simulink library "outp"  (R2021b)
(part 6 of 10)

      link override Signal_Override/_ovrdflg: Value=KOUTP_FDCBCMDVRSignalRCmd_flg_ovrdflg
      link override Signal_Override/_ovrdval: Value=KOUTP_FDCBCMDVRSignalRCmd_flg_ovrdval
  VBCM_FDCBCMEmExitSWSta_flg_Inproc : FVT_lib/outp/OverrideAndLimit  SystemSampleTime=-1  VariantActivationTime=update diagram  Latency=0  AutoFrameSizeCalculation=off
      link override Signal_Limit/_maxval: Value=KOUTP_FDCBCMEmExitSWSta_flg_maxval
      link override Signal_Limit/_minval: Value=KOUTP_FDCBCMEmExitSWSta_flg_minval
      link override Signal_Override/_ovrdflg: Value=KOUTP_FDCBCMEmExitSWSta_flg_ovrdflg
      link override Signal_Override/_ovrdval: Value=KOUTP_FDCBCMEmExitSWSta_flg_ovrdval
  VBCM_FDCBCMEmSVCmd_flg_Inproc : FVT_lib/outp/OverrideAndLimit  SystemSampleTime=-1  VariantActivationTime=update diagram  Latency=0  AutoFrameSizeCalculation=off
      link override Signal_Limit/_maxval: Value=KOUTP_FDCBCMEmSVCmd_flg_maxval
      link override Signal_Limit/_minval: Value=KOUTP_FDCBCMEmSVCmd_flg_minval
      link override Signal_Override/_ovrdflg: Value=KOUTP_FDCBCMEmSVCmd_flg_ovrdflg
      link override Signal_Override/_ovrdval: Value=KOUTP_FDCBCMEmSVCmd_flg_ovrdval
  VBCM_FDCBCMFDCloseSVCmd_flg_Inproc : FVT_lib/outp/OverrideAndLimit  SystemSampleTime=-1  VariantActivationTime=update diagram  Latency=0  AutoFrameSizeCalculation=off
      link override Signal_Limit/_maxval: Value=KOUTP_FDCBCMFDCloseSVCmd_flg_maxval
      link override Signal_Limit/_minval: Value=KOUTP_FDCBCMFDCloseSVCmd_flg_minval
      link override Signal_Override/_ovrdflg: Value=KOUTP_FDCBCMFDCloseSVCmd_flg_ovrdflg
      link override Signal_Override/_ovrdval: Value=KOUTP_FDCBCMFDCloseSVCmd_flg_ovrdval
  VBCM_FDCBCMFDOpenSVCmd_flg_Inproc : FVT_lib/outp/OverrideAndLimit  SystemSampleTime=-1  VariantActivationTime=update diagram  Latency=0  AutoFrameSizeCalculation=off
      link override Signal_Limit/_maxval: Value=KOUTP_FDCBCMFDOpenSVCmd_flg_maxval
      link override Signal_Limit/_minval: Value=KOUTP_FDCBCMFDOpenSVCmd_flg_minval
      link override Signal_Override/_ovrdflg: Value=KOUTP_FDCBCMFDOpenSVCmd_flg_ovrdflg
      link override Signal_Override/_ovrdval: Value=KOUTP_FDCBCMFDOpenSVCmd_flg_ovrdval
  VBCM_FDCBCMFDoorSta_flg_Inproc : FVT_lib/outp/OverrideAndLimit  SystemSampleTime=-1  VariantActivationTime=update diagram  Latency=0  AutoFrameSizeCalculation=off
      link override Signal_Limit/_maxval: Value=KOUTP_FDCBCMFDoorSta_flg_maxval
      link override Signal_Limit/_minval: Value=KOUTP_FDCBCMFDoorSta_flg_minval
      link override Signal_Override/_ovrdflg: Value=KOUTP_FDCBCMFDoorSta_flg_ovrdflg
      link override Signal_Override/_ovrdval: Value=KOUTP_FDCBCMFDoorSta_flg_ovrdval
  VBCM_FDCBCMFRoomLpCmd_pct_Inproc : FVT_lib/outp/OverrideAndLimit  SystemSampleTime=-1  VariantActivationTime=update diagram  Latency=0  AutoFrameSizeCalculation=off
      link override Signal_Limit/_maxval: Value=KOUTP_FDCBCMFRoomLpCmd_pct_maxval
      link override Signal_Limit/_minval: Value=KOUTP_FDCBCMFRoomLpCmd_pct_minval
      link override Signal_Override/_ovrdflg: Value=KOUTP_FDCBCMFRoomLpCmd_pct_ovrdflg
      link override Signal_Override/_ovrdval: Value=KOUTP_FDCBCMFRoomLpCmd_pct_ovrdval
  VBCM_FDCBCMFRoomLpSetSta_pct_Inproc : FVT_lib/outp/OverrideAndLimit  SystemSampleTime=-1  VariantActivationTime=update diagram  Latency=0  AutoFrameSizeCalculation=off
      link override Signal_Limit/_maxval: Value=KOUTP_FDCBCMFRoomLpSetSta_pct_maxval
      link override Signal_Limit/_minval: Value=KOUTP_FDCBCMFRoomLpSetSta_pct_minval
      link override Signal_Override/_ovrdflg: Value=KOUTP_FDCBCMFRoomLpSetSta_pct_ovrdflg
      link override Signal_Override/_ovrdval: Value=KOUTP_FDCBCMFRoomLpSetSta_pct_ovrdval
  VBCM_FDCBCMHBeamCmd_flg_Inproc : FVT_lib/outp/OverrideAndLimit  SystemSampleTime=-1  VariantActivationTime=update diagram  Latency=0  AutoFrameSizeCalculation=off
      link override Signal_Limit/_maxval: Value=KOUTP_FDCBCMHBeamCmd_flg_maxval
      link override Signal_Limit/_minval: Value=KOUTP_FDCBCMHBeamCmd_flg_minval
      link override Signal_Override/_ovrdflg: Value=KOUTP_FDCBCMHBeamCmd_flg_ovrdflg
      link override Signal_Override/_ovrdval: Value=KOUTP_FDCBCMHBeamCmd_flg_ovrdval
  VBCM_FDCBCMHelpINDCmd_flg_Inproc : FVT_lib/outp/OverrideAndLimit  SystemSampleTime=-1  VariantActivationTime=update diagram  Latency=0  AutoFrameSizeCalculation=off
      link override Signal_Limit/_maxval: Value=KOUTP_FDCBCMHelpINDCmd_flg_maxval
      link override Signal_Limit/_minval: Value=KOUTP_FDCBCMHelpINDCmd_flg_minval
      link override Signal_Override/_ovrdflg: Value=KOUTP_FDCBCMHelpINDCmd_flg_ovrdflg
      link override Signal_Override/_ovrdval: Value=KOUTP_FDCBCMHelpINDCmd_flg_ovrdval
  VBCM_FDCBCMInnerBuzzerCmd_flg_Inproc : FVT_lib/outp/OverrideAndLimit  SystemSampleTime=-1  VariantActivationTime=update diagram  Latency=0  AutoFrameSizeCalculation=off
      link override Signal_Limit/_maxval: Value=KOUTP_FDCBCMInnerBuzzerCmd_flg_maxval
      link override Signal_Limit/_minval: Value=KOUTP_FDCBCMInnerBuzzerCmd_flg_minval
      link override Signal_Override/_ovrdflg: Value=KOUTP_FDCBCMInnerBuzzerCmd_flg_ovrdflg
      link override Signal_Override/_ovrdval: Value=KOUTP_FDCBCMInnerBuzzerCmd_flg_ovrdval
  VBCM_FDCBCMInnerCallBellCmd_flg_Inproc : FVT_lib/outp/OverrideAndLimit  SystemSampleTime=-1  VariantActivationTime=update diagram  Latency=0  AutoFrameSizeCalculation=off
      link override Signal_Limit/_maxval: Value=KOUTP_FDCBCMInnerCallBellCmd_flg_maxval
      link override Signal_Limit/_minval: Value=KOUTP_FDCBCMInnerCallBellCmd_flg_minval
      link override Signal_Override/_ovrdflg: Value=KOUTP_FDCBCMInnerCallBellCmd_flg_ovrdflg
      link override Signal_Override/_ovrdval: Value=KOUTP_FDCBCMInnerCallBellCmd_flg_ovrdval
  VBCM_FDCBCMLBSDRCmd_flg_Inproc : FVT_lib/outp/OverrideAndLimit  SystemSampleTime=-1  VariantActivationTime=update diagram  Latency=0  AutoFrameSizeCalculation=off
      link override Signal_Limit/_maxval: Value=KOUTP_FDCBCMLBSDRCmd_flg_maxval
      link override Signal_Limit/_minval: Value=KOUTP_FDCBCMLBSDRCmd_flg_minval
      link override Signal_Override/_ovrdflg: Value=KOUTP_FDCBCMLBSDRCmd_flg_ovrdflg
      link override Signal_Override/_ovrdval: Value=KOUTP_FDCBCMLBSDRCmd_flg_ovrdval
  VBCM_FDCBCMLBSDYCmd_flg_Inproc : FVT_lib/outp/OverrideAndLimit  SystemSampleTime=-1  VariantActivationTime=update diagram  Latency=0  AutoFrameSizeCalculation=off
      link override Signal_Limit/_maxval: Value=KOUTP_FDCBCMLBSDYCmd_flg_maxval
      link override Signal_Limit/_minval: Value=KOUTP_FDCBCMLBSDYCmd_flg_minval
      link override Signal_Override/_ovrdflg: Value=KOUTP_FDCBCMLBSDYCmd_flg_ovrdflg
      link override Signal_Override/_ovrdval: Value=KOUTP_FDCBCMLBSDYCmd_flg_ovrdval
  VBCM_FDCBCMLBeamCmd_flg_Inproc : FVT_lib/outp/OverrideAndLimit  SystemSampleTime=-1  VariantActivationTime=update diagram  Latency=0  AutoFrameSizeCalculation=off
      link override Signal_Limit/_maxval: Value=KOUTP_FDCBCMLBeamCmd_flg_maxval
      link override Signal_Limit/_minval: Value=KOUTP_FDCBCMLBeamCmd_flg_minval
      link override Signal_Override/_ovrdflg: Value=KOUTP_FDCBCMLBeamCmd_flg_ovrdflg
      link override Signal_Override/_ovrdval: Value=KOUTP_FDCBCMLBeamCmd_flg_ovrdval
  VBCM_FDCBCMLDRLCmd_flg_Inproc : FVT_lib/outp/OverrideAndLimit  SystemSampleTime=-1  VariantActivationTime=update diagram  Latency=0  AutoFrameSizeCalculation=off
      link override Signal_Limit/_maxval: Value=KOUTP_FDCBCMLDRLCmd_flg_maxval
      link override Signal_Limit/_minval: Value=KOUTP_FDCBCMLDRLCmd_flg_minval
      link override Signal_Override/_ovrdflg: Value=KOUTP_FDCBCMLDRLCmd_flg_ovrdflg
      link override Signal_Override/_ovrdval: Value=KOUTP_FDCBCMLDRLCmd_flg_ovrdval
  VBCM_FDCBCMLTurnLpCmd_flg_Inproc : FVT_lib/outp/OverrideAndLimit  SystemSampleTime=-1  VariantActivationTime=update diagram  Latency=0  AutoFrameSizeCalculation=off
      link override Signal_Limit/_maxval: Value=KOUTP_FDCBCMLTurnLpCmd_flg_maxval
      link override Signal_Limit/_minval: Value=KOUTP_FDCBCMLTurnLpCmd_flg_minval
      link override Signal_Override/_ovrdflg: Value=KOUTP_FDCBCMLTurnLpCmd_flg_ovrdflg
      link override Signal_Override/_ovrdval: Value=KOUTP_FDCBCMLTurnLpCmd_flg_ovrdval
  VBCM_FDCBCMLTurnSWSta_flg_Inproc : FVT_lib/outp/OverrideAndLimit  SystemSampleTime=-1  VariantActivationTime=update diagram  Latency=0  AutoFrameSizeCalculation=off
      link override Signal_Limit/_maxval: Value=KOUTP_FDCBCMLTurnSWSta_flg_maxval
      link override Signal_Limit/_minval: Value=KOUTP_FDCBCMLTurnSWSta_flg_minval
      link override Signal_Override/_ovrdflg: Value=KOUTP_FDCBCMLTurnSWSta_flg_ovrdflg
      link override Signal_Override/_ovrdval: Value=KOUTP_FDCBCMLTurnSWSta_flg_ovrdval
  VBCM_FDCBCMMDCloseSVCmd_flg_Inproc : FVT_lib/outp/OverrideAndLimit  SystemSampleTime=-1  VariantActivationTime=update diagram  Latency=0  AutoFrameSizeCalculation=off
      link override Signal_Limit/_maxval: Value=KOUTP_FDCBCMMDCloseSVCmd_flg_maxval
      link override Signal_Limit/_minval: Value=KOUTP_FDCBCMMDCloseSVCmd_flg_minval
      link override Signal_Override/_ovrdflg: Value=KOUTP_FDCBCMMDCloseSVCmd_flg_ovrdflg
      link override Signal_Override/_ovrdval: Value=KOUTP_FDCBCMMDCloseSVCmd_flg_ovrdval
  VBCM_FDCBCMMDOpenSVCmd_flg_Inproc : FVT_lib/outp/OverrideAndLimit  SystemSampleTime=-1  VariantActivationTime=update diagram  Latency=0  AutoFrameSizeCalculation=off
      link override Signal_Limit/_maxval: Value=KOUTP_FDCBCMMDOpenSVCmd_flg_maxval
      link override Signal_Limit/_minval: Value=KOUTP_FDCBCMMDOpenSVCmd_flg_minval
      link override Signal_Override/_ovrdflg: Value=KOUTP_FDCBCMMDOpenSVCmd_flg_ovrdflg
      link override Signal_Override/_ovrdval: Value=KOUTP_FDCBCMMDOpenSVCmd_flg_ovrdval
  VBCM_FDCBCMMDoorSta_flg_Inproc : FVT_lib/outp/OverrideAndLimit  SystemSampleTime=-1  VariantActivationTime=update diagram  Latency=0  AutoFrameSizeCalculation=off
      link override Signal_Limit/_maxval: Value=KOUTP_FDCBCMMDoorSta_flg_maxval
      link override Signal_Limit/_minval: Value=KOUTP_FDCBCMMDoorSta_flg_minval
      link override Signal_Override/_ovrdflg: Value=KOUTP_FDCBCMMDoorSta_flg_ovrdflg
      link override Signal_Override/_ovrdval: Value=KOUTP_FDCBCMMDoorSta_flg_ovrdval
  VBCM_FDCBCMMRoomLpCmd_pct_Inproc : FVT_lib/outp/OverrideAndLimit  SystemSampleTime=-1  VariantActivationTime=update diagram  Latency=0  AutoFrameSizeCalculation=off
      link override Signal_Limit/_maxval: Value=KOUTP_FDCBCMMRoomLpCmd_pct_maxval
      link override Signal_Limit/_minval: Value=KOUTP_FDCBCMMRoomLpCmd_pct_minval
      link override Signal_Override/_ovrdflg: Value=KOUTP_FDCBCMMRoomLpCmd_pct_ovrdflg
      link override Signal_Override/_ovrdval: Value=KOUTP_FDCBCMMRoomLpCmd_pct_ovrdval
  VBCM_FDCBCMMRoomLpSetSta_pct_Inproc : FVT_lib/outp/OverrideAndLimit  SystemSampleTime=-1  VariantActivationTime=update diagram  Latency=0  AutoFrameSizeCalculation=off
      link override Signal_Limit/_maxval: Value=KOUTP_FDCBCMMRoomLpSetSta_pct_maxval
      link override Signal_Limit/_minval: Value=KOUTP_FDCBCMMRoomLpSetSta_pct_minval
      link override Signal_Override/_ovrdflg: Value=KOUTP_FDCBCMMRoomLpSetSta_pct_ovrdflg
      link override Signal_Override/_ovrdval: Value=KOUTP_FDCBCMMRoomLpSetSta_pct_ovrdval
  VBCM_FDCBCMOSDrOpenSWSta_enum_Inproc : FVT_lib/outp/OverrideAndLimit  SystemSampleTime=-1  VariantActivationTime=update diagram  Latency=0  AutoFrameSizeCalculation=off
      link override Signal_Limit/_maxval: Value=KOUTP_FDCBCMOSDrOpenSWSta_enum_maxval
      link override Signal_Limit/_minval: Value=KOUTP_FDCBCMOSDrOpenSWSta_enum_minval
      link override Signal_Override/_ovrdflg: Value=KOUTP_FDCBCMOSDrOpenSWSta_enum_ovrdflg
      link override Signal_Override/_ovrdval: Value=KOUTP_FDCBCMOSDrOpenSWSta_enum_ovrdval
  VBCM_FDCBCMPLampCmd_flg_Inproc : FVT_lib/outp/OverrideAndLimit  SystemSampleTime=-1  VariantActivationTime=update diagram  Latency=0  AutoFrameSizeCalculation=off
      link override Signal_Limit/_maxval: Value=KOUTP_FDCBCMPLampCmd_flg_maxval
      link override Signal_Limit/_minval: Value=KOUTP_FDCBCMPLampCmd_flg_minval
      link override Signal_Override/_ovrdflg: Value=KOUTP_FDCBCMPLampCmd_flg_ovrdflg
      link override Signal_Override/_ovrdval: Value=KOUTP_FDCBCMPLampCmd_flg_ovrdval
  VBCM_FDCBCMRBSDRCmd_flg_Inproc : FVT_lib/outp/OverrideAndLimit  SystemSampleTime=-1  VariantActivationTime=update diagram  Latency=0  AutoFrameSizeCalculation=off
      link override Signal_Limit/_maxval: Value=KOUTP_FDCBCMRBSDRCmd_flg_maxval
      link override Signal_Limit/_minval: Value=KOUTP_FDCBCMRBSDRCmd_flg_minval
      link override Signal_Override/_ovrdflg: Value=KOUTP_FDCBCMRBSDRCmd_flg_ovrdflg
      link override Signal_Override/_ovrdval: Value=KOUTP_FDCBCMRBSDRCmd_flg_ovrdval
  VBCM_FDCBCMRBSDYCmd_flg_Inproc : FVT_lib/outp/OverrideAndLimit  SystemSampleTime=-1  VariantActivationTime=update diagram  Latency=0  AutoFrameSizeCalculation=off
      link override Signal_Limit/_maxval: Value=KOUTP_FDCBCMRBSDYCmd_flg_maxval
      link override Signal_Limit/_minval: Value=KOUTP_FDCBCMRBSDYCmd_flg_minval
      link override Signal_Override/_ovrdflg: Value=KOUTP_FDCBCMRBSDYCmd_flg_ovrdflg
      link override Signal_Override/_ovrdval: Value=KOUTP_FDCBCMRBSDYCmd_flg_ovrdval
  VBCM_FDCBCMRDRLCmd_flg_Inproc : FVT_lib/outp/OverrideAndLimit  SystemSampleTime=-1  VariantActivationTime=update diagram  Latency=0  AutoFrameSizeCalculation=off
      link override Signal_Limit/_maxval: Value=KOUTP_FDCBCMRDRLCmd_flg_maxval
      link override Signal_Limit/_minval: Value=KOUTP_FDCBCMRDRLCmd_flg_minval
      link override Signal_Override/_ovrdflg: Value=KOUTP_FDCBCMRDRLCmd_flg_ovrdflg
      link override Signal_Override/_ovrdval: Value=KOUTP_FDCBCMRDRLCmd_flg_ovrdval
  VBCM_FDCBCMRDoorSta_flg_Inproc : FVT_lib/outp/OverrideAndLimit  SystemSampleTime=-1  VariantActivationTime=update diagram  Latency=0  AutoFrameSizeCalculation=off
      link override Signal_Limit/_maxval: Value=KOUTP_FDCBCMRDoorSta_flg_maxval
      link override Signal_Limit/_minval: Value=KOUTP_FDCBCMRDoorSta_flg_minval
      link override Signal_Override/_ovrdflg: Value=KOUTP_FDCBCMRDoorSta_flg_ovrdflg
      link override Signal_Override/_ovrdval: Value=KOUTP_FDCBCMRDoorSta_flg_ovrdval
  VBCM_FDCBCMRFLampCmd_flg_Inproc : FVT_lib/outp/OverrideAndLimit  SystemSampleTime=-1  VariantActivationTime=update diagram  Latency=0  AutoFrameSizeCalculation=off
      link override Signal_Limit/_maxval: Value=KOUTP_FDCBCMRFLampCmd_flg_maxval
      link override Signal_Limit/_minval: Value=KOUTP_FDCBCMRFLampCmd_flg_minval
      link override Signal_Override/_ovrdflg: Value=KOUTP_FDCBCMRFLampCmd_flg_ovrdflg
      link override Signal_Override/_ovrdval: Value=KOUTP_FDCBCMRFLampCmd_flg_ovrdval
  VBCM_FDCBCMRGearSta_flg_Inproc : FVT_lib/outp/OverrideAndLimit  SystemSampleTime=-1  VariantActivationTime=update diagram  Latency=0  AutoFrameSizeCalculation=off
      link override Signal_Limit/_maxval: Value=KOUTP_FDCBCMRGearSta_flg_maxval
      link override Signal_Limit/_minval: Value=KOUTP_FDCBCMRGearSta_flg_minval
      link override Signal_Override/_ovrdflg: Value=KOUTP_FDCBCMRGearSta_flg_ovrdflg
      link override Signal_Override/_ovrdval: Value=KOUTP_FDCBCMRGearSta_flg_ovrdval
  VBCM_FDCBCMRRoomLpCmd_pct_Inproc : FVT_lib/outp/OverrideAndLimit  SystemSampleTime=-1  VariantActivationTime=update diagram  Latency=0  AutoFrameSizeCalculation=off
      link override Signal_Limit/_maxval: Value=KOUTP_FDCBCMRRoomLpCmd_pct_maxval
      link override Signal_Limit/_minval: Value=KOUTP_FDCBCMRRoomLpCmd_pct_minval
      link override Signal_Override/_ovrdflg: Value=KOUTP_FDCBCMRRoomLpCmd_pct_ovrdflg
      link override Signal_Override/_ovrdval: Value=KOUTP_FDCBCMRRoomLpCmd_pct_ovrdval
  VBCM_FDCBCMRRoomLpSetSta_pct_Inproc : FVT_lib/outp/OverrideAndLimit  SystemSampleTime=-1  VariantActivationTime=update diagram  Latency=0  AutoFrameSizeCalculation=off
      link override Signal_Limit/_maxval: Value=KOUTP_FDCBCMRRoomLpSetSta_pct_maxval
      link override Signal_Limit/_minval: Value=KOUTP_FDCBCMRRoomLpSetSta_pct_minval
      link override Signal_Override/_ovrdflg: Value=KOUTP_FDCBCMRRoomLpSetSta_pct_ovrdflg
      link override Signal_Override/_ovrdval: Value=KOUTP_FDCBCMRRoomLpSetSta_pct_ovrdval
  VBCM_FDCBCMRTurnLpCmd_flg_Inproc : FVT_lib/outp/OverrideAndLimit  SystemSampleTime=-1  VariantActivationTime=update diagram  Latency=0  AutoFrameSizeCalculation=off
      link override Signal_Limit/_maxval: Value=KOUTP_FDCBCMRTurnLpCmd_flg_maxval
      link override Signal_Limit/_minval: Value=KOUTP_FDCBCMRTurnLpCmd_flg_minval
      link override Signal_Override/_ovrdflg: Value=KOUTP_FDCBCMRTurnLpCmd_flg_ovrdflg
      link override Signal_Override/_ovrdval: Value=KOUTP_FDCBCMRTurnLpCmd_flg_ovrdval
  VBCM_FDCBCMRTurnSWSta_flg_Inproc : FVT_lib/outp/OverrideAndLimit  SystemSampleTime=-1  VariantActivationTime=update diagram  Latency=0  AutoFrameSizeCalculation=off
      link override Signal_Limit/_maxval: Value=KOUTP_FDCBCMRTurnSWSta_flg_maxval
      link override Signal_Limit/_minval: Value=KOUTP_FDCBCMRTurnSWSta_flg_minval
      link override Signal_Override/_ovrdflg: Value=KOUTP_FDCBCMRTurnSWSta_flg_ovrdflg
      link override Signal_Override/_ovrdval: Value=KOUTP_FDCBCMRTurnSWSta_flg_ovrdval
  VBCM_FDCBCMRoomLpAmbCmd_flg_Inproc : FVT_lib/outp/OverrideAndLimit  SystemSampleTime=-1  VariantActivationTime=update diagram  Latency=0  AutoFrameSizeCalculation=off
      link override Signal_Limit/_maxval: Value=KOUTP_FDCBCMRoomLpAmbCmd_flg_maxval
      link override Signal_Limit/_minval: Value=KOUTP_FDCBCMRoomLpAmbCmd_flg_minval
      link override Signal_Override/_ovrdflg: Value=KOUTP_FDCBCMRoomLpAmbCmd_flg_ovrdflg
      link override Signal_Override/_ovrdval: Value=KOUTP_FDCBCMRoomLpAmbCmd_flg_ovrdval
  VBCM_FDCBCMRoomLpAmbSetSta_flg_Inproc : FVT_lib/outp/OverrideAndLimit  SystemSampleTime=-1  VariantActivationTime=update diagram  Latency=0  AutoFrameSizeCalculation=off
      link override Signal_Limit/_maxval: Value=KOUTP_FDCBCMRoomLpAmbSetSta_flg_maxval
      link override Signal_Limit/_minval: Value=KOUTP_FDCBCMRoomLpAmbSetSta_flg_minval
      link override Signal_Override/_ovrdflg: Value=KOUTP_FDCBCMRoomLpAmbSetSta_flg_ovrdflg
      link override Signal_Override/_ovrdval: Value=KOUTP_FDCBCMRoomLpAmbSetSta_flg_ovrdval
  VBCM_FDCBCMRoomLpSetSta_flg_Inproc : FVT_lib/outp/OverrideAndLimit  SystemSampleTime=-1  VariantActivationTime=update diagram  Latency=0  AutoFrameSizeCalculation=off
      link override Signal_Limit/_maxval: Value=KOUTP_FDCBCMRoomLpSetSta_flg_maxval
      link override Signal_Limit/_minval: Value=KOUTP_FDCBCMRoomLpSetSta_flg_minval
      link override Signal_Override/_ovrdflg: Value=KOUTP_FDCBCMRoomLpSetSta_flg_ovrdflg
      link override Signal_Override/_ovrdval: Value=KOUTP_FDCBCMRoomLpSetSta_flg_ovrdval
  VBCM_FDCBCMSLTLpCmd_flg_Inproc : FVT_lib/outp/OverrideAndLimit  SystemSampleTime=-1  VariantActivationTime=update diagram  Latency=0  AutoFrameSizeCalculation=off
      link override Signal_Limit/_maxval: Value=KOUTP_FDCBCMSLTLpCmd_flg_maxval
      link override Signal_Limit/_minval: Value=KOUTP_FDCBCMSLTLpCmd_flg_minval
      link override Signal_Override/_ovrdflg: Value=KOUTP_FDCBCMSLTLpCmd_flg_ovrdflg
      link override Signal_Override/_ovrdval: Value=KOUTP_FDCBCMSLTLpCmd_flg_ovrdval
  VBCM_FDCBCMSMKLCmd_flg_Inproc : FVT_lib/outp/OverrideAndLimit  SystemSampleTime=-1  VariantActivationTime=update diagram  Latency=0  AutoFrameSizeCalculation=off
      link override Signal_Limit/_maxval: Value=KOUTP_FDCBCMSMKLCmd_flg_maxval
      link override Signal_Limit/_minval: Value=KOUTP_FDCBCMSMKLCmd_flg_minval
      link override Signal_Override/_ovrdflg: Value=KOUTP_FDCBCMSMKLCmd_flg_ovrdflg
      link override Signal_Override/_ovrdval: Value=KOUTP_FDCBCMSMKLCmd_flg_ovrdval
  VBCM_FDCBCMSMKRCmd_flg_Inproc : FVT_lib/outp/OverrideAndLimit  SystemSampleTime=-1  VariantActivationTime=update diagram  Latency=0  AutoFrameSizeCalculation=off
      link override Signal_Limit/_maxval: Value=KOUTP_FDCBCMSMKRCmd_flg_maxval
      link override Signal_Limit/_minval: Value=KOUTP_FDCBCMSMKRCmd_flg_minval
      link override Signal_Override/_ovrdflg: Value=KOUTP_FDCBCMSMKRCmd_flg_ovrdflg
      link override Signal_Override/_ovrdval: Value=KOUTP_FDCBCMSMKRCmd_flg_ovrdval
  VBCM_FDCBCMSRTLpCmd_flg_Inproc : FVT_lib/outp/OverrideAndLimit  SystemSampleTime=-1  VariantActivationTime=update diagram  Latency=0  AutoFrameSizeCalculation=off
      link override Signal_Limit/_maxval: Value=KOUTP_FDCBCMSRTLpCmd_flg_maxval
      link override Signal_Limit/_minval: Value=KOUTP_FDCBCMSRTLpCmd_flg_minval
      link override Signal_Override/_ovrdflg: Value=KOUTP_FDCBCMSRTLpCmd_flg_ovrdflg
      link override Signal_Override/_ovrdval: Value=KOUTP_FDCBCMSRTLpCmd_flg_ovrdval
  VBCM_FDCBCMSTOPBALLCmd_flg_Inproc : FVT_lib/outp/OverrideAndLimit  SystemSampleTime=-1  VariantActivationTime=update diagram  Latency=0  AutoFrameSizeCalculation=off
      link override Signal_Limit/_maxval: Value=KOUTP_FDCBCMSTOPBALLCmd_flg_maxval
      link override Signal_Limit/_minval: Value=KOUTP_FDCBCMSTOPBALLCmd_flg_minval
      link override Signal_Override/_ovrdflg: Value=KOUTP_FDCBCMSTOPBALLCmd_flg_ovrdflg
      link override Signal_Override/_ovrdval: Value=KOUTP_FDCBCMSTOPBALLCmd_flg_ovrdval
  VBCM_FDCBCMStopINDCmd_flg_Inproc : FVT_lib/outp/OverrideAndLimit  SystemSampleTime=-1  VariantActivationTime=update diagram  Latency=0  AutoFrameSizeCalculation=off
      link override Signal_Limit/_maxval: Value=KOUTP_FDCBCMStopINDCmd_flg_maxval
      link override Signal_Limit/_minval: Value=KOUTP_FDCBCMStopINDCmd_flg_minval
      link override Signal_Override/_ovrdflg: Value=KOUTP_FDCBCMStopINDCmd_flg_ovrdflg
      link override Signal_Override/_ovrdval: Value=KOUTP_FDCBCMStopINDCmd_flg_ovrdval
  VBCM_FDCBCMTurnBuzzerENSta_flg_Inproc : FVT_lib/outp/OverrideAndLimit  SystemSampleTime=-1  VariantActivationTime=update diagram  Latency=0  AutoFrameSizeCalculation=off
      link override Signal_Limit/_maxval: Value=KOUTP_FDCBCMTurnBuzzerENSta_flg_maxval
      link override Signal_Limit/_minval: Value=KOUTP_FDCBCMTurnBuzzerENSta_flg_minval
      link override Signal_Override/_ovrdflg: Value=KOUTP_FDCBCMTurnBuzzerENSta_flg_ovrdflg
      link override Signal_Override/_ovrdval: Value=KOUTP_FDCBCMTurnBuzzerENSta_flg_ovrdval
  VBCM_FDCBCMWasherCmd_flg_Inproc : FVT_lib/outp/OverrideAndLimit  SystemSampleTime=-1  VariantActivationTime=update diagram  Latency=0  AutoFrameSizeCalculation=off
      link override Signal_Limit/_maxval: Value=KOUTP_FDCBCMWasherCmd_flg_maxval
      link override Signal_Limit/_minval: Value=KOUTP_FDCBCMWasherCmd_flg_minval
      link override Signal_Override/_ovrdflg: Value=KOUTP_FDCBCMWasherCmd_flg_ovrdflg
      link override Signal_Override/_ovrdval: Value=KOUTP_FDCBCMWasherCmd_flg_ovrdval
  VBCM_FDCBCMWiperHCmd_flg_Inproc : FVT_lib/outp/OverrideAndLimit  SystemSampleTime=-1  VariantActivationTime=update diagram  Latency=0  AutoFrameSizeCalculation=off
      link override Signal_Limit/_maxval: Value=KOUTP_FDCBCMWiperHCmd_flg_maxval
      link override Signal_Limit/_minval: Value=KOUTP_FDCBCMWiperHCmd_flg_minval
      link override Signal_Override/_ovrdflg: Value=KOUTP_FDCBCMWiperHCmd_flg_ovrdflg
      link override Signal_Override/_ovrdval: Value=KOUTP_FDCBCMWiperHCmd_flg_ovrdval
  VBCM_FDCBCMWiperLCmd_flg_Inproc : FVT_lib/outp/OverrideAndLimit  SystemSampleTime=-1  VariantActivationTime=update diagram  Latency=0  AutoFrameSizeCalculation=off
      link override Signal_Limit/_maxval: Value=KOUTP_FDCBCMWiperLCmd_flg_maxval
      link override Signal_Limit/_minval: Value=KOUTP_FDCBCMWiperLCmd_flg_minval
      link override Signal_Override/_ovrdflg: Value=KOUTP_FDCBCMWiperLCmd_flg_ovrdflg
      link override Signal_Override/_ovrdval: Value=KOUTP_FDCBCMWiperLCmd_flg_ovrdval
  VBCM_InnerBuzzerModeSta_enum_Inproc : FVT_lib/outp/OverrideAndLimit  SystemSampleTime=-1  VariantActivationTime=update diagram  Latency=0  AutoFrameSizeCalculation=off
      link override Signal_Limit/_maxval: Value=KOUTP_InnerBuzzerModeSta_enum_maxval
      link override Signal_Limit/_minval: Value=KOUTP_InnerBuzzerModeSta_enum_minval
      link override Signal_Override/_ovrdflg: Value=KOUTP_InnerBuzzerModeSta_enum_ovrdflg
      link override Signal_Override/_ovrdval: Value=KOUTP_InnerBuzzerModeSta_enum_ovrdval
  VBCM_KeepWakeUp_flg_Inproc : FVT_lib/outp/OverrideAndLimit  SystemSampleTime=-1  VariantActivationTime=update diagram  Latency=0  AutoFrameSizeCalculation=off
      link override Signal_Limit/_maxval: Value=KOUTP_KeepWakeUp_flg_maxval
      link override Signal_Limit/_minval: Value=KOUTP_KeepWakeUp_flg_minval
      link override Signal_Override/_ovrdflg: Value=KOUTP_KeepWakeUp_flg_ovrdflg
      link override Signal_Override/_ovrdval: Value=KOUTP_KeepWakeUp_flg_ovrdval
  VBCM_TurnLpPatternSta_enum_Inproc : FVT_lib/outp/OverrideAndLimit  SystemSampleTime=-1  VariantActivationTime=update diagram  Latency=0  AutoFrameSizeCalculation=off
      link override Signal_Limit/_maxval: Value=KOUTP_TurnLpPatternSta_enum_maxval
      link override Signal_Limit/_minval: Value=KOUTP_TurnLpPatternSta_enum_minval
      link override Signal_Override/_ovrdflg: Value=KOUTP_TurnLpPatternSta_enum_ovrdflg
      link override Signal_Override/_ovrdval: Value=KOUTP_TurnLpPatternSta_enum_ovrdval
  VBCM_WakeUp_flg_Inproc : FVT_lib/outp/OverrideAndLimit  SystemSampleTime=-1  VariantActivationTime=update diagram  Latency=0  AutoFrameSizeCalculation=off
      link override Signal_Limit/_maxval: Value=KOUTP_WakeUp_flg_maxval
      link override Signal_Limit/_minval: Value=KOUTP_WakeUp_flg_minval
      link override Signal_Override/_ovrdflg: Value=KOUTP_WakeUp_flg_ovrdflg
      link override Signal_Override/_ovrdval: Value=KOUTP_WakeUp_flg_ovrdval
  VDDM_5vAPS1PwrErrDTC_raw32_Inproc : FVT_lib/outp/OverrideAndLimit  SystemSampleTime=-1  VariantActivationTime=update diagram  Latency=0  AutoFrameSizeCalculation=off
      link override Signal_Limit/_maxval: Value=KOUTP_5vAPS1PwrErrDTC_raw32_maxval
      link override Signal_Limit/_minval: Value=KOUTP_5vAPS1PwrErrDTC_raw32_minval
      link override Signal_Override/_ovrdflg: Value=KOUTP_5vAPS1PwrErrDTC_raw32_ovrdflg
      link override Signal_Override/_ovrdval: Value=KOUTP_5vAPS1PwrErrDTC_raw32_ovrdval
  VDDM_5vAPS2PwrErrDTC_raw32_Inproc : FVT_lib/outp/OverrideAndLimit  SystemSampleTime=-1  VariantActivationTime=update diagram  Latency=0  AutoFrameSizeCalculation=off
      link override Signal_Limit/_maxval: Value=KOUTP_5vAPS2PwrErrDTC_raw32_maxval
      link override Signal_Limit/_minval: Value=KOUTP_5vAPS2PwrErrDTC_raw32_minval
      link override Signal_Override/_ovrdflg: Value=KOUTP_5vAPS2PwrErrDTC_raw32_ovrdflg
      link override Signal_Override/_ovrdval: Value=KOUTP_5vAPS2PwrErrDTC_raw32_ovrdval
  VDDM_ACCAccelCmdErrDetDTC_raw32_Inproc : FVT_lib/outp/OverrideAndLimit  SystemSampleTime=-1  VariantActivationTime=update diagram  Latency=0  AutoFrameSizeCalculation=off
      link override Signal_Limit/_maxval: Value=KOUTP_ACCAccelCmdErrDetDTC_raw32_maxval
      link override Signal_Limit/_minval: Value=KOUTP_ACCAccelCmdErrDetDTC_raw32_minval
      link override Signal_Override/_ovrdflg: Value=KOUTP_ACCAccelCmdErrDetDTC_raw32_ovrdflg
      link override Signal_Override/_ovrdval: Value=KOUTP_ACCAccelCmdErrDetDTC_raw32_ovrdval
  VDDM_ACCMalfuncDetDTC_raw32_Inproc : FVT_lib/outp/OverrideAndLimit  SystemSampleTime=-1  VariantActivationTime=update diagram  Latency=0  AutoFrameSizeCalculation=off
      link override Signal_Limit/_maxval: Value=KOUTP_ACCMalfuncDetDTC_raw32_maxval
      link override Signal_Limit/_minval: Value=KOUTP_ACCMalfuncDetDTC_raw32_minval
      link override Signal_Override/_ovrdflg: Value=KOUTP_ACCMalfuncDetDTC_raw32_ovrdflg
      link override Signal_Override/_ovrdval: Value=KOUTP_ACCMalfuncDetDTC_raw32_ovrdval
  VDDM_APS1SigOoRDTC_raw32_Inproc : FVT_lib/outp/OverrideAndLimit  SystemSampleTime=-1  VariantActivationTime=update diagram  Latency=0  AutoFrameSizeCalculation=off
      link override Signal_Limit/_maxval: Value=KOUTP_APS1SigOoRDTC_raw32_maxval
      link override Signal_Limit/_minval: Value=KOUTP_APS1SigOoRDTC_raw32_minval
      link override Signal_Override/_ovrdflg: Value=KOUTP_APS1SigOoRDTC_raw32_ovrdflg
      link override Signal_Override/_ovrdval: Value=KOUTP_APS1SigOoRDTC_raw32_ovrdval
  VDDM_APS2SigOoRDTC_raw32_Inproc : FVT_lib/outp/OverrideAndLimit  SystemSampleTime=-1  VariantActivationTime=update diagram  Latency=0  AutoFrameSizeCalculation=off
      link override Signal_Limit/_maxval: Value=KOUTP_APS2SigOoRDTC_raw32_maxval
      link override Signal_Limit/_minval: Value=KOUTP_APS2SigOoRDTC_raw32_minval
      link override Signal_Override/_ovrdflg: Value=KOUTP_APS2SigOoRDTC_raw32_ovrdflg
      link override Signal_Override/_ovrdval: Value=KOUTP_APS2SigOoRDTC_raw32_ovrdval
  VDDM_APSCorrErrDTC_raw32_Inproc : FVT_lib/outp/OverrideAndLimit  SystemSampleTime=-1  VariantActivationTime=update diagram  Latency=0  AutoFrameSizeCalculation=off
      link override Signal_Limit/_maxval: Value=KOUTP_APSCorrErrDTC_raw32_maxval
      link override Signal_Limit/_minval: Value=KOUTP_APSCorrErrDTC_raw32_minval
      link override Signal_Override/_ovrdflg: Value=KOUTP_APSCorrErrDTC_raw32_ovrdflg
      link override Signal_Override/_ovrdval: Value=KOUTP_APSCorrErrDTC_raw32_ovrdval
  VDDM_BMSRdyDTC_raw32_Inproc : FVT_lib/outp/OverrideAndLimit  SystemSampleTime=-1  VariantActivationTime=update diagram  Latency=0  AutoFrameSizeCalculation=off
      link override Signal_Limit/_maxval: Value=KOUTP_BMSRdyDTC_raw32_maxval
      link override Signal_Limit/_minval: Value=KOUTP_BMSRdyDTC_raw32_minval
      link override Signal_Override/_ovrdflg: Value=KOUTP_BMSRdyDTC_raw32_ovrdflg
      link override Signal_Override/_ovrdval: Value=KOUTP_BMSRdyDTC_raw32_ovrdval
  VDDM_BMSSigErrDetDTC_raw32_Inproc : FVT_lib/outp/OverrideAndLimit  SystemSampleTime=-1  VariantActivationTime=update diagram  Latency=0  AutoFrameSizeCalculation=off
      link override Signal_Limit/_maxval: Value=KOUTP_BMSSigErrDetDTC_raw32_maxval
      link override Signal_Limit/_minval: Value=KOUTP_BMSSigErrDetDTC_raw32_minval
      link override Signal_Override/_ovrdflg: Value=KOUTP_BMSSigErrDetDTC_raw32_ovrdflg
      link override Signal_Override/_ovrdval: Value=KOUTP_BMSSigErrDetDTC_raw32_ovrdval
  VDDM_BrkSWErrDTC_raw32_Inproc : FVT_lib/outp/OverrideAndLimit  SystemSampleTime=-1  VariantActivationTime=update diagram  Latency=0  AutoFrameSizeCalculation=off
      link override Signal_Limit/_maxval: Value=KOUTP_BrkSWErrDTC_raw32_maxval
      link override Signal_Limit/_minval: Value=KOUTP_BrkSWErrDTC_raw32_minval
      link override Signal_Override/_ovrdflg: Value=KOUTP_BrkSWErrDTC_raw32_ovrdflg
      link override Signal_Override/_ovrdval: Value=KOUTP_BrkSWErrDTC_raw32_ovrdval
  VDDM_BrkSWNoBacDTC_raw32_Inproc : FVT_lib/outp/OverrideAndLimit  SystemSampleTime=-1  VariantActivationTime=update diagram  Latency=0  AutoFrameSizeCalculation=off
      link override Signal_Limit/_maxval: Value=KOUTP_BrkSWNoBacDTC_raw32_maxval
      link override Signal_Limit/_minval: Value=KOUTP_BrkSWNoBacDTC_raw32_minval
      link override Signal_Override/_ovrdflg: Value=KOUTP_BrkSWNoBacDTC_raw32_ovrdflg
      link override Signal_Override/_ovrdval: Value=KOUTP_BrkSWNoBacDTC_raw32_ovrdval
  VDDM_C1ABM1CSDTC_raw32_Inproc : FVT_lib/outp/OverrideAndLimit  SystemSampleTime=-1  VariantActivationTime=update diagram  Latency=0  AutoFrameSizeCalculation=off
      link override Signal_Limit/_maxval: Value=KOUTP_C1ABM1CSDTC_raw32_maxval
      link override Signal_Limit/_minval: Value=KOUTP_C1ABM1CSDTC_raw32_minval
      link override Signal_Override/_ovrdflg: Value=KOUTP_C1ABM1CSDTC_raw32_ovrdflg
      link override Signal_Override/_ovrdval: Value=KOUTP_C1ABM1CSDTC_raw32_ovrdval
  VDDM_C1ABM1LCDTC_raw32_Inproc : FVT_lib/outp/OverrideAndLimit  SystemSampleTime=-1  VariantActivationTime=update diagram  Latency=0  AutoFrameSizeCalculation=off
      link override Signal_Limit/_maxval: Value=KOUTP_C1ABM1LCDTC_raw32_maxval
      link override Signal_Limit/_minval: Value=KOUTP_C1ABM1LCDTC_raw32_minval
      link override Signal_Override/_ovrdflg: Value=KOUTP_C1ABM1LCDTC_raw32_ovrdflg
      link override Signal_Override/_ovrdval: Value=KOUTP_C1ABM1LCDTC_raw32_ovrdval
  VDDM_C1ABM1RCDTC_raw32_Inproc : FVT_lib/outp/OverrideAndLimit  SystemSampleTime=-1  VariantActivationTime=update diagram  Latency=0  AutoFrameSizeCalculation=off
      link override Signal_Limit/_maxval: Value=KOUTP_C1ABM1RCDTC_raw32_maxval
      link override Signal_Limit/_minval: Value=KOUTP_C1ABM1RCDTC_raw32_minval
      link override Signal_Override/_ovrdflg: Value=KOUTP_C1ABM1RCDTC_raw32_ovrdflg
      link override Signal_Override/_ovrdval: Value=KOUTP_C1ABM1RCDTC_raw32_ovrdval
  VDDM_C1EPAS2LCDTC_raw32_Inproc : FVT_lib/outp/OverrideAndLimit  SystemSampleTime=-1  VariantActivationTime=update diagram  Latency=0  AutoFrameSizeCalculation=off
      link override Signal_Limit/_maxval: Value=KOUTP_C1EPAS2LCDTC_raw32_maxval
      link override Signal_Limit/_minval: Value=KOUTP_C1EPAS2LCDTC_raw32_minval
      link override Signal_Override/_ovrdflg: Value=KOUTP_C1EPAS2LCDTC_raw32_ovrdflg
      link override Signal_Override/_ovrdval: Value=KOUTP_C1EPAS2LCDTC_raw32_ovrdval
  VDDM_C3BMS1CSDTC_raw32_Inproc : FVT_lib/outp/OverrideAndLimit  SystemSampleTime=-1  VariantActivationTime=update diagram  Latency=0  AutoFrameSizeCalculation=off
      link override Signal_Limit/_maxval: Value=KOUTP_C3BMS1CSDTC_raw32_maxval
      link override Signal_Limit/_minval: Value=KOUTP_C3BMS1CSDTC_raw32_minval
      link override Signal_Override/_ovrdflg: Value=KOUTP_C3BMS1CSDTC_raw32_ovrdflg
      link override Signal_Override/_ovrdval: Value=KOUTP_C3BMS1CSDTC_raw32_ovrdval
  VDDM_C3BMS1LCDTC_raw32_Inproc : FVT_lib/outp/OverrideAndLimit  SystemSampleTime=-1  VariantActivationTime=update diagram  Latency=0  AutoFrameSizeCalculation=off
      link override Signal_Limit/_maxval: Value=KOUTP_C3BMS1LCDTC_raw32_maxval
      link override Signal_Limit/_minval: Value=KOUTP_C3BMS1LCDTC_raw32_minval
      link override Signal_Override/_ovrdflg: Value=KOUTP_C3BMS1LCDTC_raw32_ovrdflg
      link override Signal_Override/_ovrdval: Value=KOUTP_C3BMS1LCDTC_raw32_ovrdval
  VDDM_C3BMS1RCDTC_raw32_Inproc : FVT_lib/outp/OverrideAndLimit  SystemSampleTime=-1  VariantActivationTime=update diagram  Latency=0  AutoFrameSizeCalculation=off
      link override Signal_Limit/_maxval: Value=KOUTP_C3BMS1RCDTC_raw32_maxval
      link override Signal_Limit/_minval: Value=KOUTP_C3BMS1RCDTC_raw32_minval
      link override Signal_Override/_ovrdflg: Value=KOUTP_C3BMS1RCDTC_raw32_ovrdflg
      link override Signal_Override/_ovrdval: Value=KOUTP_C3BMS1RCDTC_raw32_ovrdval
  VDDM_C3BMS6CSDTC_raw32_Inproc : FVT_lib/outp/OverrideAndLimit  SystemSampleTime=-1  VariantActivationTime=update diagram  Latency=0  AutoFrameSizeCalculation=off
      link override Signal_Limit/_maxval: Value=KOUTP_C3BMS6CSDTC_raw32_maxval
      link override Signal_Limit/_minval: Value=KOUTP_C3BMS6CSDTC_raw32_minval
      link override Signal_Override/_ovrdflg: Value=KOUTP_C3BMS6CSDTC_raw32_ovrdflg
      link override Signal_Override/_ovrdval: Value=KOUTP_C3BMS6CSDTC_raw32_ovrdval
  VDDM_C3BMS6LCDTC_raw32_Inproc : FVT_lib/outp/OverrideAndLimit  SystemSampleTime=-1  VariantActivationTime=update diagram  Latency=0  AutoFrameSizeCalculation=off
      link override Signal_Limit/_maxval: Value=KOUTP_C3BMS6LCDTC_raw32_maxval
      link override Signal_Limit/_minval: Value=KOUTP_C3BMS6LCDTC_raw32_minval
      link override Signal_Override/_ovrdflg: Value=KOUTP_C3BMS6LCDTC_raw32_ovrdflg
      link override Signal_Override/_ovrdval: Value=KOUTP_C3BMS6LCDTC_raw32_ovrdval
  VDDM_C3BMS6RCDTC_raw32_Inproc : FVT_lib/outp/OverrideAndLimit  SystemSampleTime=-1  VariantActivationTime=update diagram  Latency=0  AutoFrameSizeCalculation=off
      link override Signal_Limit/_maxval: Value=KOUTP_C3BMS6RCDTC_raw32_maxval
      link override Signal_Limit/_minval: Value=KOUTP_C3BMS6RCDTC_raw32_minval
      link override Signal_Override/_ovrdflg: Value=KOUTP_C3BMS6RCDTC_raw32_ovrdflg
      link override Signal_Override/_ovrdval: Value=KOUTP_C3BMS6RCDTC_raw32_ovrdval
  VDDM_C3CCU1CSDTC_raw32_Inproc : FVT_lib/outp/OverrideAndLimit  SystemSampleTime=-1  VariantActivationTime=update diagram  Latency=0  AutoFrameSizeCalculation=off
      link override Signal_Limit/_maxval: Value=KOUTP_C3CCU1CSDTC_raw32_maxval
      link override Signal_Limit/_minval: Value=KOUTP_C3CCU1CSDTC_raw32_minval
      link override Signal_Override/_ovrdflg: Value=KOUTP_C3CCU1CSDTC_raw32_ovrdflg
      link override Signal_Override/_ovrdval: Value=KOUTP_C3CCU1CSDTC_raw32_ovrdval
  VDDM_C3CCU1LCDTC_raw32_Inproc : FVT_lib/outp/OverrideAndLimit  SystemSampleTime=-1  VariantActivationTime=update diagram  Latency=0  AutoFrameSizeCalculation=off
      link override Signal_Limit/_maxval: Value=KOUTP_C3CCU1LCDTC_raw32_maxval
      link override Signal_Limit/_minval: Value=KOUTP_C3CCU1LCDTC_raw32_minval
      link override Signal_Override/_ovrdflg: Value=KOUTP_C3CCU1LCDTC_raw32_ovrdflg
      link override Signal_Override/_ovrdval: Value=KOUTP_C3CCU1LCDTC_raw32_ovrdval
  VDDM_C3CCU1RCDTC_raw32_Inproc : FVT_lib/outp/OverrideAndLimit  SystemSampleTime=-1  VariantActivationTime=update diagram  Latency=0  AutoFrameSizeCalculation=off
      link override Signal_Limit/_maxval: Value=KOUTP_C3CCU1RCDTC_raw32_maxval
      link override Signal_Limit/_minval: Value=KOUTP_C3CCU1RCDTC_raw32_minval
      link override Signal_Override/_ovrdflg: Value=KOUTP_C3CCU1RCDTC_raw32_ovrdflg
      link override Signal_Override/_ovrdval: Value=KOUTP_C3CCU1RCDTC_raw32_ovrdval
  VDDM_C3CCU2CSDTC_raw32_Inproc : FVT_lib/outp/OverrideAndLimit  SystemSampleTime=-1  VariantActivationTime=update diagram  Latency=0  AutoFrameSizeCalculation=off
      link override Signal_Limit/_maxval: Value=KOUTP_C3CCU2CSDTC_raw32_maxval
      link override Signal_Limit/_minval: Value=KOUTP_C3CCU2CSDTC_raw32_minval
      link override Signal_Override/_ovrdflg: Value=KOUTP_C3CCU2CSDTC_raw32_ovrdflg
      link override Signal_Override/_ovrdval: Value=KOUTP_C3CCU2CSDTC_raw32_ovrdval
  VDDM_C3CCU2LCDTC_raw32_Inproc : FVT_lib/outp/OverrideAndLimit  SystemSampleTime=-1  VariantActivationTime=update diagram  Latency=0  AutoFrameSizeCalculation=off
      link override Signal_Limit/_maxval: Value=KOUTP_C3CCU2LCDTC_raw32_maxval
      link override Signal_Limit/_minval: Value=KOUTP_C3CCU2LCDTC_raw32_minval
      link override Signal_Override/_ovrdflg: Value=KOUTP_C3CCU2LCDTC_raw32_ovrdflg
      link override Signal_Override/_ovrdval: Value=KOUTP_C3CCU2LCDTC_raw32_ovrdval
  VDDM_C3CCU2RCDTC_raw32_Inproc : FVT_lib/outp/OverrideAndLimit  SystemSampleTime=-1  VariantActivationTime=update diagram  Latency=0  AutoFrameSizeCalculation=off
      link override Signal_Limit/_maxval: Value=KOUTP_C3CCU2RCDTC_raw32_maxval
      link override Signal_Limit/_minval: Value=KOUTP_C3CCU2RCDTC_raw32_minval
      link override Signal_Override/_ovrdflg: Value=KOUTP_C3CCU2RCDTC_raw32_ovrdflg
      link override Signal_Override/_ovrdval: Value=KOUTP_C3CCU2RCDTC_raw32_ovrdval
  VDDM_CCMalfuncDetDTC_raw32_Inproc : FVT_lib/outp/OverrideAndLimit  SystemSampleTime=-1  VariantActivationTime=update diagram  Latency=0  AutoFrameSizeCalculation=off
      link override Signal_Limit/_maxval: Value=KOUTP_CCMalfuncDetDTC_raw32_maxval
      link override Signal_Limit/_minval: Value=KOUTP_CCMalfuncDetDTC_raw32_minval
      link override Signal_Override/_ovrdflg: Value=KOUTP_CCMalfuncDetDTC_raw32_ovrdflg
      link override Signal_Override/_ovrdval: Value=KOUTP_CCMalfuncDetDTC_raw32_ovrdval
  VDDM_CCUSigErrDetDTC_raw32_Inproc : FVT_lib/outp/OverrideAndLimit  SystemSampleTime=-1  VariantActivationTime=update diagram  Latency=0  AutoFrameSizeCalculation=off
      link override Signal_Limit/_maxval: Value=KOUTP_CCUSigErrDetDTC_raw32_maxval
      link override Signal_Limit/_minval: Value=KOUTP_CCUSigErrDetDTC_raw32_minval
      link override Signal_Override/_ovrdflg: Value=KOUTP_CCUSigErrDetDTC_raw32_ovrdflg
      link override Signal_Override/_ovrdval: Value=KOUTP_CCUSigErrDetDTC_raw32_ovrdval
  VDDM_DCDC4PreDTC_raw32_Inproc : FVT_lib/outp/OverrideAndLimit  SystemSampleTime=-1  VariantActivationTime=update diagram  Latency=0  AutoFrameSizeCalculation=off
      link override Signal_Limit/_maxval: Value=KOUTP_DCDC4PreDTC_raw32_maxval
      link override Signal_Limit/_minval: Value=KOUTP_DCDC4PreDTC_raw32_minval
      link override Signal_Override/_ovrdflg: Value=KOUTP_DCDC4PreDTC_raw32_ovrdflg
      link override Signal_Override/_ovrdval: Value=KOUTP_DCDC4PreDTC_raw32_ovrdval
  VDDM_DCDCDisDTC_raw32_Inproc : FVT_lib/outp/OverrideAndLimit  SystemSampleTime=-1  VariantActivationTime=update diagram  Latency=0  AutoFrameSizeCalculation=off
      link override Signal_Limit/_maxval: Value=KOUTP_DCDCDisDTC_raw32_maxval
      link override Signal_Limit/_minval: Value=KOUTP_DCDCDisDTC_raw32_minval
      link override Signal_Override/_ovrdflg: Value=KOUTP_DCDCDisDTC_raw32_ovrdflg
      link override Signal_Override/_ovrdval: Value=KOUTP_DCDCDisDTC_raw32_ovrdval
  VDDM_DCDCEnaDTC_raw32_Inproc : FVT_lib/outp/OverrideAndLimit  SystemSampleTime=-1  VariantActivationTime=update diagram  Latency=0  AutoFrameSizeCalculation=off
      link override Signal_Limit/_maxval: Value=KOUTP_DCDCEnaDTC_raw32_maxval
      link override Signal_Limit/_minval: Value=KOUTP_DCDCEnaDTC_raw32_minval
      link override Signal_Override/_ovrdflg: Value=KOUTP_DCDCEnaDTC_raw32_ovrdflg
      link override Signal_Override/_ovrdval: Value=KOUTP_DCDCEnaDTC_raw32_ovrdval
  VDDM_DTCDetect_enum_Inproc : FVT_lib/outp/OverrideAndLimit  SystemSampleTime=-1  VariantActivationTime=update diagram  Latency=0  AutoFrameSizeCalculation=off
      link override Signal_Limit/_maxval: Value=KOUTP_DTCDetect_enum_maxval
      link override Signal_Limit/_minval: Value=KOUTP_DTCDetect_enum_minval
      link override Signal_Override/_ovrdflg: Value=KOUTP_DTCDetect_enum_ovrdflg
      link override Signal_Override/_ovrdval: Value=KOUTP_DTCDetect_enum_ovrdval
  VDDM_DiagFLTSDTC_raw32_Inproc : FVT_lib/outp/OverrideAndLimit  SystemSampleTime=-1  VariantActivationTime=update diagram  Latency=0  AutoFrameSizeCalculation=off
      link override Signal_Limit/_maxval: Value=KOUTP_DiagFLTSDTC_raw32_maxval
      link override Signal_Limit/_minval: Value=KOUTP_DiagFLTSDTC_raw32_minval
      link override Signal_Override/_ovrdflg: Value=KOUTP_DiagFLTSDTC_raw32_ovrdflg
      link override Signal_Override/_ovrdval: Value=KOUTP_DiagFLTSDTC_raw32_ovrdval
  VDDM_DiagFRTSDTC_raw32_Inproc : FVT_lib/outp/OverrideAndLimit  SystemSampleTime=-1  VariantActivationTime=update diagram  Latency=0  AutoFrameSizeCalculation=off
      link override Signal_Limit/_maxval: Value=KOUTP_DiagFRTSDTC_raw32_maxval
      link override Signal_Limit/_minval: Value=KOUTP_DiagFRTSDTC_raw32_minval
      link override Signal_Override/_ovrdflg: Value=KOUTP_DiagFRTSDTC_raw32_ovrdflg
      link override Signal_Override/_ovrdval: Value=KOUTP_DiagFRTSDTC_raw32_ovrdval
  VDDM_DiagHCrashDTC_raw32_Inproc : FVT_lib/outp/OverrideAndLimit  SystemSampleTime=-1  VariantActivationTime=update diagram  Latency=0  AutoFrameSizeCalculation=off
      link override Signal_Limit/_maxval: Value=KOUTP_DiagHCrashDTC_raw32_maxval
      link override Signal_Limit/_minval: Value=KOUTP_DiagHCrashDTC_raw32_minval
      link override Signal_Override/_ovrdflg: Value=KOUTP_DiagHCrashDTC_raw32_ovrdflg
      link override Signal_Override/_ovrdval: Value=KOUTP_DiagHCrashDTC_raw32_ovrdval
  VDDM_DiagRLTSDTC_raw32_Inproc : FVT_lib/outp/OverrideAndLimit  SystemSampleTime=-1  VariantActivationTime=update diagram  Latency=0  AutoFrameSizeCalculation=off
      link override Signal_Limit/_maxval: Value=KOUTP_DiagRLTSDTC_raw32_maxval
      link override Signal_Limit/_minval: Value=KOUTP_DiagRLTSDTC_raw32_minval
      link override Signal_Override/_ovrdflg: Value=KOUTP_DiagRLTSDTC_raw32_ovrdflg
      link override Signal_Override/_ovrdval: Value=KOUTP_DiagRLTSDTC_raw32_ovrdval
  VDDM_DiagRRTSDTC_raw32_Inproc : FVT_lib/outp/OverrideAndLimit  SystemSampleTime=-1  VariantActivationTime=update diagram  Latency=0  AutoFrameSizeCalculation=off
      link override Signal_Limit/_maxval: Value=KOUTP_DiagRRTSDTC_raw32_maxval
      link override Signal_Limit/_minval: Value=KOUTP_DiagRRTSDTC_raw32_minval
      link override Signal_Override/_ovrdflg: Value=KOUTP_DiagRRTSDTC_raw32_ovrdflg
      link override Signal_Override/_ovrdval: Value=KOUTP_DiagRRTSDTC_raw32_ovrdval
  VDDM_DisengagePFail_flg_Inproc : FVT_lib/outp/OverrideAndLimit  SystemSampleTime=-1  VariantActivationTime=update diagram  Latency=0  AutoFrameSizeCalculation=off
      link override Signal_Limit/_maxval: Value=KOUTP_DisengagePFail_flg_maxval
      link override Signal_Limit/_minval: Value=KOUTP_DisengagePFail_flg_minval
      link override Signal_Override/_ovrdflg: Value=KOUTP_DisengagePFail_flg_ovrdflg
      link override Signal_Override/_ovrdval: Value=KOUTP_DisengagePFail_flg_ovrdval
  VDDM_DrStSWDTC_raw32_Inproc : FVT_lib/outp/OverrideAndLimit  SystemSampleTime=-1  VariantActivationTime=update diagram  Latency=0  AutoFrameSizeCalculation=off
      link override Signal_Limit/_maxval: Value=KOUTP_DrStSWDTC_raw32_maxval
      link override Signal_Limit/_minval: Value=KOUTP_DrStSWDTC_raw32_minval
      link override Signal_Override/_ovrdflg: Value=KOUTP_DrStSWDTC_raw32_ovrdflg
      link override Signal_Override/_ovrdval: Value=KOUTP_DrStSWDTC_raw32_ovrdval
  VDDM_EDriveSysErrShifterErr_flg_Inproc : FVT_lib/outp/OverrideAndLimit  SystemSampleTime=-1  VariantActivationTime=update diagram  Latency=0  AutoFrameSizeCalculation=off
      link override Signal_Limit/_maxval: Value=KOUTP_EDriveSysErrShifterErr_flg_maxval
      link override Signal_Limit/_minval: Value=KOUTP_EDriveSysErrShifterErr_flg_minval
      link override Signal_Override/_ovrdflg: Value=KOUTP_EDriveSysErrShifterErr_flg_ovrdflg
      link override Signal_Override/_ovrdval: Value=KOUTP_EDriveSysErrShifterErr_flg_ovrdval
  VDDM_EDriveSysErrVCUErr_flg_Inproc : FVT_lib/outp/OverrideAndLimit  SystemSampleTime=-1  VariantActivationTime=update diagram  Latency=0  AutoFrameSizeCalculation=off
      link override Signal_Limit/_maxval: Value=KOUTP_EDriveSysErrVCUErr_flg_maxval
      link override Signal_Limit/_minval: Value=KOUTP_EDriveSysErrVCUErr_flg_minval
      link override Signal_Override/_ovrdflg: Value=KOUTP_EDriveSysErrVCUErr_flg_ovrdflg
      link override Signal_Override/_ovrdval: Value=KOUTP_EDriveSysErrVCUErr_flg_ovrdval
  VDDM_EPBLockTODTC_raw32_Inproc : FVT_lib/outp/OverrideAndLimit  SystemSampleTime=-1  VariantActivationTime=update diagram  Latency=0  AutoFrameSizeCalculation=off
      link override Signal_Limit/_maxval: Value=KOUTP_EPBLockTODTC_raw32_maxval
      link override Signal_Limit/_minval: Value=KOUTP_EPBLockTODTC_raw32_minval
      link override Signal_Override/_ovrdflg: Value=KOUTP_EPBLockTODTC_raw32_ovrdflg
      link override Signal_Override/_ovrdval: Value=KOUTP_EPBLockTODTC_raw32_ovrdval
  VDDM_EPBUnlockTODTC_raw32_Inproc : FVT_lib/outp/OverrideAndLimit  SystemSampleTime=-1  VariantActivationTime=update diagram  Latency=0  AutoFrameSizeCalculation=off
      link override Signal_Limit/_maxval: Value=KOUTP_EPBUnlockTODTC_raw32_maxval
      link override Signal_Limit/_minval: Value=KOUTP_EPBUnlockTODTC_raw32_minval
      link override Signal_Override/_ovrdflg: Value=KOUTP_EPBUnlockTODTC_raw32_ovrdflg
      link override Signal_Override/_ovrdval: Value=KOUTP_EPBUnlockTODTC_raw32_ovrdval
  VDDM_ESC1CSErrDTC_raw32_Inproc : FVT_lib/outp/OverrideAndLimit  SystemSampleTime=-1  VariantActivationTime=update diagram  Latency=0  AutoFrameSizeCalculation=off
      link override Signal_Limit/_maxval: Value=KOUTP_ESC1CSErrDTC_raw32_maxval
      link override Signal_Limit/_minval: Value=KOUTP_ESC1CSErrDTC_raw32_minval
      link override Signal_Override/_ovrdflg: Value=KOUTP_ESC1CSErrDTC_raw32_ovrdflg
      link override Signal_Override/_ovrdval: Value=KOUTP_ESC1CSErrDTC_raw32_ovrdval
  VDDM_ESC1NoComDTC_raw32_Inproc : FVT_lib/outp/OverrideAndLimit  SystemSampleTime=-1  VariantActivationTime=update diagram  Latency=0  AutoFrameSizeCalculation=off
      link override Signal_Limit/_maxval: Value=KOUTP_ESC1NoComDTC_raw32_maxval
      link override Signal_Limit/_minval: Value=KOUTP_ESC1NoComDTC_raw32_minval
      link override Signal_Override/_ovrdflg: Value=KOUTP_ESC1NoComDTC_raw32_ovrdflg
      link override Signal_Override/_ovrdval: Value=KOUTP_ESC1NoComDTC_raw32_ovrdval
  VDDM_ESC1RCErrDTC_raw32_Inproc : FVT_lib/outp/OverrideAndLimit  SystemSampleTime=-1  VariantActivationTime=update diagram  Latency=0  AutoFrameSizeCalculation=off
      link override Signal_Limit/_maxval: Value=KOUTP_ESC1RCErrDTC_raw32_maxval
      link override Signal_Limit/_minval: Value=KOUTP_ESC1RCErrDTC_raw32_minval
      link override Signal_Override/_ovrdflg: Value=KOUTP_ESC1RCErrDTC_raw32_ovrdflg
      link override Signal_Override/_ovrdval: Value=KOUTP_ESC1RCErrDTC_raw32_ovrdval
  VDDM_ESC5CSErrDTC_raw32_Inproc : FVT_lib/outp/OverrideAndLimit  SystemSampleTime=-1  VariantActivationTime=update diagram  Latency=0  AutoFrameSizeCalculation=off
      link override Signal_Limit/_maxval: Value=KOUTP_ESC5CSErrDTC_raw32_maxval
      link override Signal_Limit/_minval: Value=KOUTP_ESC5CSErrDTC_raw32_minval
      link override Signal_Override/_ovrdflg: Value=KOUTP_ESC5CSErrDTC_raw32_ovrdflg
      link override Signal_Override/_ovrdval: Value=KOUTP_ESC5CSErrDTC_raw32_ovrdval
  VDDM_ESC5NoComDTC_raw32_Inproc : FVT_lib/outp/OverrideAndLimit  SystemSampleTime=-1  VariantActivationTime=update diagram  Latency=0  AutoFrameSizeCalculation=off
      link override Signal_Limit/_maxval: Value=KOUTP_ESC5NoComDTC_raw32_maxval
      link override Signal_Limit/_minval: Value=KOUTP_ESC5NoComDTC_raw32_minval
      link override Signal_Override/_ovrdflg: Value=KOUTP_ESC5NoComDTC_raw32_ovrdflg
      link override Signal_Override/_ovrdval: Value=KOUTP_ESC5NoComDTC_raw32_ovrdval
  VDDM_ESC5RCErrDTC_raw32_Inproc : FVT_lib/outp/OverrideAndLimit  SystemSampleTime=-1  VariantActivationTime=update diagram  Latency=0  AutoFrameSizeCalculation=off
      link override Signal_Limit/_maxval: Value=KOUTP_ESC5RCErrDTC_raw32_maxval
      link override Signal_Limit/_minval: Value=KOUTP_ESC5RCErrDTC_raw32_minval
      link override Signal_Override/_ovrdflg: Value=KOUTP_ESC5RCErrDTC_raw32_ovrdflg
      link override Signal_Override/_ovrdval: Value=KOUTP_ESC5RCErrDTC_raw32_ovrdval
  VDDM_ESC7CSErrDTC_raw32_Inproc : FVT_lib/outp/OverrideAndLimit  SystemSampleTime=-1  VariantActivationTime=update diagram  Latency=0  AutoFrameSizeCalculation=off
      link override Signal_Limit/_maxval: Value=KOUTP_ESC7CSErrDTC_raw32_maxval
      link override Signal_Limit/_minval: Value=KOUTP_ESC7CSErrDTC_raw32_minval
      link override Signal_Override/_ovrdflg: Value=KOUTP_ESC7CSErrDTC_raw32_ovrdflg
      link override Signal_Override/_ovrdval: Value=KOUTP_ESC7CSErrDTC_raw32_ovrdval
  VDDM_ESC7NoComDTC_raw32_Inproc : FVT_lib/outp/OverrideAndLimit  SystemSampleTime=-1  VariantActivationTime=update diagram  Latency=0  AutoFrameSizeCalculation=off
      link override Signal_Limit/_maxval: Value=KOUTP_ESC7NoComDTC_raw32_maxval
      link override Signal_Limit/_minval: Value=KOUTP_ESC7NoComDTC_raw32_minval
      link override Signal_Override/_ovrdflg: Value=KOUTP_ESC7NoComDTC_raw32_ovrdflg
      link override Signal_Override/_ovrdval: Value=KOUTP_ESC7NoComDTC_raw32_ovrdval
  VDDM_ESC7RCErrDTC_raw32_Inproc : FVT_lib/outp/OverrideAndLimit  SystemSampleTime=-1  VariantActivationTime=update diagram  Latency=0  AutoFrameSizeCalculation=off
      link override Signal_Limit/_maxval: Value=KOUTP_ESC7RCErrDTC_raw32_maxval
      link override Signal_Limit/_minval: Value=KOUTP_ESC7RCErrDTC_raw32_minval
      link override Signal_Override/_ovrdflg: Value=KOUTP_ESC7RCErrDTC_raw32_ovrdflg
      link override Signal_Override/_ovrdval: Value=KOUTP_ESC7RCErrDTC_raw32_ovrdval
  VDDM_EngagePFail_flg_Inproc : FVT_lib/outp/OverrideAndLimit  SystemSampleTime=-1  VariantActivationTime=update diagram  Latency=0  AutoFrameSizeCalculation=off
      link override Signal_Limit/_maxval: Value=KOUTP_EngagePFail_flg_maxval
      link override Signal_Limit/_minval: Value=KOUTP_EngagePFail_flg_minval
      link override Signal_Override/_ovrdflg: Value=KOUTP_EngagePFail_flg_ovrdflg
      link override Signal_Override/_ovrdval: Value=KOUTP_EngagePFail_flg_ovrdval
  VDDM_EnterNewOperCyc_flg_Inproc : FVT_lib/outp/OverrideAndLimit  SystemSampleTime=-1  VariantActivationTime=update diagram  Latency=0  AutoFrameSizeCalculation=off
      link override Signal_Limit/_maxval: Value=KOUTP_EnterNewOperCyc_flg_maxval
      link override Signal_Limit/_minval: Value=KOUTP_EnterNewOperCyc_flg_minval
      link override Signal_Override/_ovrdflg: Value=KOUTP_EnterNewOperCyc_flg_ovrdflg
      link override Signal_Override/_ovrdval: Value=KOUTP_EnterNewOperCyc_flg_ovrdval
  VDDM_FCLUSSDTC_raw32_Inproc : FVT_lib/outp/OverrideAndLimit  SystemSampleTime=-1  VariantActivationTime=update diagram  Latency=0  AutoFrameSizeCalculation=off
      link override Signal_Limit/_maxval: Value=KOUTP_FCLUSSDTC_raw32_maxval
      link override Signal_Limit/_minval: Value=KOUTP_FCLUSSDTC_raw32_minval
      link override Signal_Override/_ovrdflg: Value=KOUTP_FCLUSSDTC_raw32_ovrdflg
      link override Signal_Override/_ovrdval: Value=KOUTP_FCLUSSDTC_raw32_ovrdval
  VDDM_FCM2CSErrDTC_raw32_Inproc : FVT_lib/outp/OverrideAndLimit  SystemSampleTime=-1  VariantActivationTime=update diagram  Latency=0  AutoFrameSizeCalculation=off
      link override Signal_Limit/_maxval: Value=KOUTP_FCM2CSErrDTC_raw32_maxval
      link override Signal_Limit/_minval: Value=KOUTP_FCM2CSErrDTC_raw32_minval
      link override Signal_Override/_ovrdflg: Value=KOUTP_FCM2CSErrDTC_raw32_ovrdflg
      link override Signal_Override/_ovrdval: Value=KOUTP_FCM2CSErrDTC_raw32_ovrdval
  VDDM_FCM2NoComDTC_raw32_Inproc : FVT_lib/outp/OverrideAndLimit  SystemSampleTime=-1  VariantActivationTime=update diagram  Latency=0  AutoFrameSizeCalculation=off
      link override Signal_Limit/_maxval: Value=KOUTP_FCM2NoComDTC_raw32_maxval
      link override Signal_Limit/_minval: Value=KOUTP_FCM2NoComDTC_raw32_minval
      link override Signal_Override/_ovrdflg: Value=KOUTP_FCM2NoComDTC_raw32_ovrdflg
      link override Signal_Override/_ovrdval: Value=KOUTP_FCM2NoComDTC_raw32_ovrdval
  VDDM_FCM2RCErrDTC_raw32_Inproc : FVT_lib/outp/OverrideAndLimit  SystemSampleTime=-1  VariantActivationTime=update diagram  Latency=0  AutoFrameSizeCalculation=off
      link override Signal_Limit/_maxval: Value=KOUTP_FCM2RCErrDTC_raw32_maxval
      link override Signal_Limit/_minval: Value=KOUTP_FCM2RCErrDTC_raw32_minval
      link override Signal_Override/_ovrdflg: Value=KOUTP_FCM2RCErrDTC_raw32_ovrdflg
      link override Signal_Override/_ovrdval: Value=KOUTP_FCM2RCErrDTC_raw32_ovrdval
  VDDM_FCM3CSErrDTC_raw32_Inproc : FVT_lib/outp/OverrideAndLimit  SystemSampleTime=-1  VariantActivationTime=update diagram  Latency=0  AutoFrameSizeCalculation=off
      link override Signal_Limit/_maxval: Value=KOUTP_FCM3CSErrDTC_raw32_maxval
      link override Signal_Limit/_minval: Value=KOUTP_FCM3CSErrDTC_raw32_minval
      link override Signal_Override/_ovrdflg: Value=KOUTP_FCM3CSErrDTC_raw32_ovrdflg
      link override Signal_Override/_ovrdval: Value=KOUTP_FCM3CSErrDTC_raw32_ovrdval
  VDDM_FCM3NoComDTC_raw32_Inproc : FVT_lib/outp/OverrideAndLimit  SystemSampleTime=-1  VariantActivationTime=update diagram  Latency=0  AutoFrameSizeCalculation=off
      link override Signal_Limit/_maxval: Value=KOUTP_FCM3NoComDTC_raw32_maxval
      link override Signal_Limit/_minval: Value=KOUTP_FCM3NoComDTC_raw32_minval
      link override Signal_Override/_ovrdflg: Value=KOUTP_FCM3NoComDTC_raw32_ovrdflg
      link override Signal_Override/_ovrdval: Value=KOUTP_FCM3NoComDTC_raw32_ovrdval
  VDDM_FCM3RCErrDTC_raw32_Inproc : FVT_lib/outp/OverrideAndLimit  SystemSampleTime=-1  VariantActivationTime=update diagram  Latency=0  AutoFrameSizeCalculation=off
      link override Signal_Limit/_maxval: Value=KOUTP_FCM3RCErrDTC_raw32_maxval
      link override Signal_Limit/_minval: Value=KOUTP_FCM3RCErrDTC_raw32_minval
      link override Signal_Override/_ovrdflg: Value=KOUTP_FCM3RCErrDTC_raw32_ovrdflg
      link override Signal_Override/_ovrdval: Value=KOUTP_FCM3RCErrDTC_raw32_ovrdval
  VDDM_FCM4CSErrDTC_raw32_Inproc : FVT_lib/outp/OverrideAndLimit  SystemSampleTime=-1  VariantActivationTime=update diagram  Latency=0  AutoFrameSizeCalculation=off
      link override Signal_Limit/_maxval: Value=KOUTP_FCM4CSErrDTC_raw32_maxval
      link override Signal_Limit/_minval: Value=KOUTP_FCM4CSErrDTC_raw32_minval
      link override Signal_Override/_ovrdflg: Value=KOUTP_FCM4CSErrDTC_raw32_ovrdflg
      link override Signal_Override/_ovrdval: Value=KOUTP_FCM4CSErrDTC_raw32_ovrdval
  VDDM_FCM4NoComDTC_raw32_Inproc : FVT_lib/outp/OverrideAndLimit  SystemSampleTime=-1  VariantActivationTime=update diagram  Latency=0  AutoFrameSizeCalculation=off
      link override Signal_Limit/_maxval: Value=KOUTP_FCM4NoComDTC_raw32_maxval
      link override Signal_Limit/_minval: Value=KOUTP_FCM4NoComDTC_raw32_minval
      link override Signal_Override/_ovrdflg: Value=KOUTP_FCM4NoComDTC_raw32_ovrdflg
      link override Signal_Override/_ovrdval: Value=KOUTP_FCM4NoComDTC_raw32_ovrdval
  VDDM_FCM5CSErrDTC_raw32_Inproc : FVT_lib/outp/OverrideAndLimit  SystemSampleTime=-1  VariantActivationTime=update diagram  Latency=0  AutoFrameSizeCalculation=off
      link override Signal_Limit/_maxval: Value=KOUTP_FCM5CSErrDTC_raw32_maxval
      link override Signal_Limit/_minval: Value=KOUTP_FCM5CSErrDTC_raw32_minval
      link override Signal_Override/_ovrdflg: Value=KOUTP_FCM5CSErrDTC_raw32_ovrdflg
      link override Signal_Override/_ovrdval: Value=KOUTP_FCM5CSErrDTC_raw32_ovrdval
  VDDM_FCM5NoComDTC_raw32_Inproc : FVT_lib/outp/OverrideAndLimit  SystemSampleTime=-1  VariantActivationTime=update diagram  Latency=0  AutoFrameSizeCalculation=off
      link override Signal_Limit/_maxval: Value=KOUTP_FCM5NoComDTC_raw32_maxval
      link override Signal_Limit/_minval: Value=KOUTP_FCM5NoComDTC_raw32_minval
      link override Signal_Override/_ovrdflg: Value=KOUTP_FCM5NoComDTC_raw32_ovrdflg
      link override Signal_Override/_ovrdval: Value=KOUTP_FCM5NoComDTC_raw32_ovrdval
  VDDM_FCMACCSigErrDetDTC_raw32_Inproc : FVT_lib/outp/OverrideAndLimit  SystemSampleTime=-1  VariantActivationTime=update diagram  Latency=0  AutoFrameSizeCalculation=off
      link override Signal_Limit/_maxval: Value=KOUTP_FCMACCSigErrDetDTC_raw32_maxval
      link override Signal_Limit/_minval: Value=KOUTP_FCMACCSigErrDetDTC_raw32_minval
      link override Signal_Override/_ovrdflg: Value=KOUTP_FCMACCSigErrDetDTC_raw32_ovrdflg
      link override Signal_Override/_ovrdval: Value=KOUTP_FCMACCSigErrDetDTC_raw32_ovrdval
  VDDM_FCRUSSDTC_raw32_Inproc : FVT_lib/outp/OverrideAndLimit  SystemSampleTime=-1  VariantActivationTime=update diagram  Latency=0  AutoFrameSizeCalculation=off
      link override Signal_Limit/_maxval: Value=KOUTP_FCRUSSDTC_raw32_maxval
      link override Signal_Limit/_minval: Value=KOUTP_FCRUSSDTC_raw32_minval
      link override Signal_Override/_ovrdflg: Value=KOUTP_FCRUSSDTC_raw32_ovrdflg
      link override Signal_Override/_ovrdval: Value=KOUTP_FCRUSSDTC_raw32_ovrdval
  VDDM_FLDoorSWDTC_raw32_Inproc : FVT_lib/outp/OverrideAndLimit  SystemSampleTime=-1  VariantActivationTime=update diagram  Latency=0  AutoFrameSizeCalculation=off
      link override Signal_Limit/_maxval: Value=KOUTP_FLDoorSWDTC_raw32_maxval
      link override Signal_Limit/_minval: Value=KOUTP_FLDoorSWDTC_raw32_minval
      link override Signal_Override/_ovrdflg: Value=KOUTP_FLDoorSWDTC_raw32_ovrdflg
      link override Signal_Override/_ovrdval: Value=KOUTP_FLDoorSWDTC_raw32_ovrdval
  VDDM_FLLUSSDTC_raw32_Inproc : FVT_lib/outp/OverrideAndLimit  SystemSampleTime=-1  VariantActivationTime=update diagram  Latency=0  AutoFrameSizeCalculation=off
      link override Signal_Limit/_maxval: Value=KOUTP_FLLUSSDTC_raw32_maxval
      link override Signal_Limit/_minval: Value=KOUTP_FLLUSSDTC_raw32_minval
      link override Signal_Override/_ovrdflg: Value=KOUTP_FLLUSSDTC_raw32_ovrdflg
      link override Signal_Override/_ovrdval: Value=KOUTP_FLLUSSDTC_raw32_ovrdval
  VDDM_FLRUSSDTC_raw32_Inproc : FVT_lib/outp/OverrideAndLimit  SystemSampleTime=-1  VariantActivationTime=update diagram  Latency=0  AutoFrameSizeCalculation=off
      link override Signal_Limit/_maxval: Value=KOUTP_FLRUSSDTC_raw32_maxval
      link override Signal_Limit/_minval: Value=KOUTP_FLRUSSDTC_raw32_minval
      link override Signal_Override/_ovrdflg: Value=KOUTP_FLRUSSDTC_raw32_ovrdflg
      link override Signal_Override/_ovrdval: Value=KOUTP_FLRUSSDTC_raw32_ovrdval
  VDDM_FMLUSSDTC_raw32_Inproc : FVT_lib/outp/OverrideAndLimit  SystemSampleTime=-1  VariantActivationTime=update diagram  Latency=0  AutoFrameSizeCalculation=off
      link override Signal_Limit/_maxval: Value=KOUTP_FMLUSSDTC_raw32_maxval
      link override Signal_Limit/_minval: Value=KOUTP_FMLUSSDTC_raw32_minval
      link override Signal_Override/_ovrdflg: Value=KOUTP_FMLUSSDTC_raw32_ovrdflg
      link override Signal_Override/_ovrdval: Value=KOUTP_FMLUSSDTC_raw32_ovrdval
  VDDM_FMRUSSDTC_raw32_Inproc : FVT_lib/outp/OverrideAndLimit  SystemSampleTime=-1  VariantActivationTime=update diagram  Latency=0  AutoFrameSizeCalculation=off
      link override Signal_Limit/_maxval: Value=KOUTP_FMRUSSDTC_raw32_maxval
      link override Signal_Limit/_minval: Value=KOUTP_FMRUSSDTC_raw32_minval
      link override Signal_Override/_ovrdflg: Value=KOUTP_FMRUSSDTC_raw32_ovrdflg
      link override Signal_Override/_ovrdval: Value=KOUTP_FMRUSSDTC_raw32_ovrdval
  VDDM_FRDoorSWDTC_raw32_Inproc : FVT_lib/outp/OverrideAndLimit  SystemSampleTime=-1  VariantActivationTime=update diagram  Latency=0  AutoFrameSizeCalculation=off
      link override Signal_Limit/_maxval: Value=KOUTP_FRDoorSWDTC_raw32_maxval
      link override Signal_Limit/_minval: Value=KOUTP_FRDoorSWDTC_raw32_minval
      link override Signal_Override/_ovrdflg: Value=KOUTP_FRDoorSWDTC_raw32_ovrdflg
      link override Signal_Override/_ovrdval: Value=KOUTP_FRDoorSWDTC_raw32_ovrdval
  VDDM_FrMCUSigErrDetDTC_raw32_Inproc : FVT_lib/outp/OverrideAndLimit  SystemSampleTime=-1  VariantActivationTime=update diagram  Latency=0  AutoFrameSizeCalculation=off
      link override Signal_Limit/_maxval: Value=KOUTP_FrMCUSigErrDetDTC_raw32_maxval
      link override Signal_Limit/_minval: Value=KOUTP_FrMCUSigErrDetDTC_raw32_minval
      link override Signal_Override/_ovrdflg: Value=KOUTP_FrMCUSigErrDetDTC_raw32_ovrdflg
      link override Signal_Override/_ovrdval: Value=KOUTP_FrMCUSigErrDetDTC_raw32_ovrdval
  VDDM_FrMCUTqErrDTC_raw32_Inproc : FVT_lib/outp/OverrideAndLimit  SystemSampleTime=-1  VariantActivationTime=update diagram  Latency=0  AutoFrameSizeCalculation=off
      link override Signal_Limit/_maxval: Value=KOUTP_FrMCUTqErrDTC_raw32_maxval
      link override Signal_Limit/_minval: Value=KOUTP_FrMCUTqErrDTC_raw32_minval
      link override Signal_Override/_ovrdflg: Value=KOUTP_FrMCUTqErrDTC_raw32_ovrdflg
      link override Signal_Override/_ovrdval: Value=KOUTP_FrMCUTqErrDTC_raw32_ovrdval
  VDDM_HVB4PreDTC_raw32_Inproc : FVT_lib/outp/OverrideAndLimit  SystemSampleTime=-1  VariantActivationTime=update diagram  Latency=0  AutoFrameSizeCalculation=off
      link override Signal_Limit/_maxval: Value=KOUTP_HVB4PreDTC_raw32_maxval
      link override Signal_Limit/_minval: Value=KOUTP_HVB4PreDTC_raw32_minval
      link override Signal_Override/_ovrdflg: Value=KOUTP_HVB4PreDTC_raw32_ovrdflg
      link override Signal_Override/_ovrdval: Value=KOUTP_HVB4PreDTC_raw32_ovrdval
  VDDM_HVRlyCloDTC_raw32_Inproc : FVT_lib/outp/OverrideAndLimit  SystemSampleTime=-1  VariantActivationTime=update diagram  Latency=0  AutoFrameSizeCalculation=off
      link override Signal_Limit/_maxval: Value=KOUTP_HVRlyCloDTC_raw32_maxval
      link override Signal_Limit/_minval: Value=KOUTP_HVRlyCloDTC_raw32_minval
      link override Signal_Override/_ovrdflg: Value=KOUTP_HVRlyCloDTC_raw32_ovrdflg
      link override Signal_Override/_ovrdval: Value=KOUTP_HVRlyCloDTC_raw32_ovrdval
  VDDM_HVRlyOpDTC_raw32_Inproc : FVT_lib/outp/OverrideAndLimit  SystemSampleTime=-1  VariantActivationTime=update diagram  Latency=0  AutoFrameSizeCalculation=off
      link override Signal_Limit/_maxval: Value=KOUTP_HVRlyOpDTC_raw32_maxval
      link override Signal_Limit/_minval: Value=KOUTP_HVRlyOpDTC_raw32_minval
      link override Signal_Override/_ovrdflg: Value=KOUTP_HVRlyOpDTC_raw32_ovrdflg
      link override Signal_Override/_ovrdval: Value=KOUTP_HVRlyOpDTC_raw32_ovrdval
  VDDM_HVRlyOpFail_flg_Inproc : FVT_lib/outp/OverrideAndLimit  SystemSampleTime=-1  VariantActivationTime=update diagram  Latency=0  AutoFrameSizeCalculation=off
      link override Signal_Limit/_maxval: Value=KOUTP_HVRlyOpFail_flg_maxval
      link override Signal_Limit/_minval: Value=KOUTP_HVRlyOpFail_flg_minval
      link override Signal_Override/_ovrdflg: Value=KOUTP_HVRlyOpFail_flg_ovrdflg
      link override Signal_Override/_ovrdval: Value=KOUTP_HVRlyOpFail_flg_ovrdval
  VDDM_HiLvSaChkDTC_raw32_Inproc : FVT_lib/outp/OverrideAndLimit  SystemSampleTime=-1  VariantActivationTime=update diagram  Latency=0  AutoFrameSizeCalculation=off
      link override Signal_Limit/_maxval: Value=KOUTP_HiLvSaChkDTC_raw32_maxval
      link override Signal_Limit/_minval: Value=KOUTP_HiLvSaChkDTC_raw32_minval
      link override Signal_Override/_ovrdflg: Value=KOUTP_HiLvSaChkDTC_raw32_ovrdflg
      link override Signal_Override/_ovrdval: Value=KOUTP_HiLvSaChkDTC_raw32_ovrdval
  VDDM_HoodSWDTC_raw32_Inproc : FVT_lib/outp/OverrideAndLimit  SystemSampleTime=-1  VariantActivationTime=update diagram  Latency=0  AutoFrameSizeCalculation=off
      link override Signal_Limit/_maxval: Value=KOUTP_HoodSWDTC_raw32_maxval
      link override Signal_Limit/_minval: Value=KOUTP_HoodSWDTC_raw32_minval
      link override Signal_Override/_ovrdflg: Value=KOUTP_HoodSWDTC_raw32_ovrdflg
      link override Signal_Override/_ovrdval: Value=KOUTP_HoodSWDTC_raw32_ovrdval
  VDDM_ISAMalfuncDetDTC_raw32_Inproc : FVT_lib/outp/OverrideAndLimit  SystemSampleTime=-1  VariantActivationTime=update diagram  Latency=0  AutoFrameSizeCalculation=off
      link override Signal_Limit/_maxval: Value=KOUTP_ISAMalfuncDetDTC_raw32_maxval
      link override Signal_Limit/_minval: Value=KOUTP_ISAMalfuncDetDTC_raw32_minval
      link override Signal_Override/_ovrdflg: Value=KOUTP_ISAMalfuncDetDTC_raw32_ovrdflg
      link override Signal_Override/_ovrdval: Value=KOUTP_ISAMalfuncDetDTC_raw32_ovrdval
  VDDM_IniLVLoDTC_raw32_Inproc : FVT_lib/outp/OverrideAndLimit  SystemSampleTime=-1  VariantActivationTime=update diagram  Latency=0  AutoFrameSizeCalculation=off
      link override Signal_Limit/_maxval: Value=KOUTP_IniLVLoDTC_raw32_maxval
      link override Signal_Limit/_minval: Value=KOUTP_IniLVLoDTC_raw32_minval
      link override Signal_Override/_ovrdflg: Value=KOUTP_IniLVLoDTC_raw32_ovrdflg
      link override Signal_Override/_ovrdval: Value=KOUTP_IniLVLoDTC_raw32_ovrdval
  VDDM_KeyAuthDTC_raw32_Inproc : FVT_lib/outp/OverrideAndLimit  SystemSampleTime=-1  VariantActivationTime=update diagram  Latency=0  AutoFrameSizeCalculation=off
      link override Signal_Limit/_maxval: Value=KOUTP_KeyAuthDTC_raw32_maxval
      link override Signal_Limit/_minval: Value=KOUTP_KeyAuthDTC_raw32_minval
      link override Signal_Override/_ovrdflg: Value=KOUTP_KeyAuthDTC_raw32_ovrdflg
      link override Signal_Override/_ovrdval: Value=KOUTP_KeyAuthDTC_raw32_ovrdval
  VDDM_LFBatwarnDTC_raw32_Inproc : FVT_lib/outp/OverrideAndLimit  SystemSampleTime=-1  VariantActivationTime=update diagram  Latency=0  AutoFrameSizeCalculation=off
      link override Signal_Limit/_maxval: Value=KOUTP_LFBatwarnDTC_raw32_maxval
      link override Signal_Limit/_minval: Value=KOUTP_LFBatwarnDTC_raw32_minval
      link override Signal_Override/_ovrdflg: Value=KOUTP_LFBatwarnDTC_raw32_ovrdflg
      link override Signal_Override/_ovrdval: Value=KOUTP_LFBatwarnDTC_raw32_ovrdval
  VDDM_LFPressIndiDTC_raw32_Inproc : FVT_lib/outp/OverrideAndLimit  SystemSampleTime=-1  VariantActivationTime=update diagram  Latency=0  AutoFrameSizeCalculation=off
      link override Signal_Limit/_maxval: Value=KOUTP_LFPressIndiDTC_raw32_maxval
      link override Signal_Limit/_minval: Value=KOUTP_LFPressIndiDTC_raw32_minval
      link override Signal_Override/_ovrdflg: Value=KOUTP_LFPressIndiDTC_raw32_ovrdflg
      link override Signal_Override/_ovrdval: Value=KOUTP_LFPressIndiDTC_raw32_ovrdval
  VDDM_LFSensorFailDTC_raw32_Inproc : FVT_lib/outp/OverrideAndLimit  SystemSampleTime=-1  VariantActivationTime=update diagram  Latency=0  AutoFrameSizeCalculation=off
      link override Signal_Limit/_maxval: Value=KOUTP_LFSensorFailDTC_raw32_maxval
      link override Signal_Limit/_minval: Value=KOUTP_LFSensorFailDTC_raw32_minval
      link override Signal_Override/_ovrdflg: Value=KOUTP_LFSensorFailDTC_raw32_ovrdflg
      link override Signal_Override/_ovrdval: Value=KOUTP_LFSensorFailDTC_raw32_ovrdval
  VDDM_LFWheelTmpHighDTC_raw32_Inproc : FVT_lib/outp/OverrideAndLimit  SystemSampleTime=-1  VariantActivationTime=update diagram  Latency=0  AutoFrameSizeCalculation=off
      link override Signal_Limit/_maxval: Value=KOUTP_LFWheelTmpHighDTC_raw32_maxval
      link override Signal_Limit/_minval: Value=KOUTP_LFWheelTmpHighDTC_raw32_minval
      link override Signal_Override/_ovrdflg: Value=KOUTP_LFWheelTmpHighDTC_raw32_ovrdflg
      link override Signal_Override/_ovrdval: Value=KOUTP_LFWheelTmpHighDTC_raw32_ovrdval
  VDDM_LRBatwarnDTC_raw32_Inproc : FVT_lib/outp/OverrideAndLimit  SystemSampleTime=-1  VariantActivationTime=update diagram  Latency=0  AutoFrameSizeCalculation=off
      link override Signal_Limit/_maxval: Value=KOUTP_LRBatwarnDTC_raw32_maxval
      link override Signal_Limit/_minval: Value=KOUTP_LRBatwarnDTC_raw32_minval
      link override Signal_Override/_ovrdflg: Value=KOUTP_LRBatwarnDTC_raw32_ovrdflg
      link override Signal_Override/_ovrdval: Value=KOUTP_LRBatwarnDTC_raw32_ovrdval
  VDDM_LRPressIndiDTC_raw32_Inproc : FVT_lib/outp/OverrideAndLimit  SystemSampleTime=-1  VariantActivationTime=update diagram  Latency=0  AutoFrameSizeCalculation=off
      link override Signal_Limit/_maxval: Value=KOUTP_LRPressIndiDTC_raw32_maxval
      link override Signal_Limit/_minval: Value=KOUTP_LRPressIndiDTC_raw32_minval
      link override Signal_Override/_ovrdflg: Value=KOUTP_LRPressIndiDTC_raw32_ovrdflg
      link override Signal_Override/_ovrdval: Value=KOUTP_LRPressIndiDTC_raw32_ovrdval
  VDDM_LRSensorFailDTC_raw32_Inproc : FVT_lib/outp/OverrideAndLimit  SystemSampleTime=-1  VariantActivationTime=update diagram  Latency=0  AutoFrameSizeCalculation=off
      link override Signal_Limit/_maxval: Value=KOUTP_LRSensorFailDTC_raw32_maxval
      link override Signal_Limit/_minval: Value=KOUTP_LRSensorFailDTC_raw32_minval
      link override Signal_Override/_ovrdflg: Value=KOUTP_LRSensorFailDTC_raw32_ovrdflg
      link override Signal_Override/_ovrdval: Value=KOUTP_LRSensorFailDTC_raw32_ovrdval
  VDDM_LRWheelTmpHighDTC_raw32_Inproc : FVT_lib/outp/OverrideAndLimit  SystemSampleTime=-1  VariantActivationTime=update diagram  Latency=0  AutoFrameSizeCalculation=off
      link override Signal_Limit/_maxval: Value=KOUTP_LRWheelTmpHighDTC_raw32_maxval
      link override Signal_Limit/_minval: Value=KOUTP_LRWheelTmpHighDTC_raw32_minval
      link override Signal_Override/_ovrdflg: Value=KOUTP_LRWheelTmpHighDTC_raw32_ovrdflg
      link override Signal_Override/_ovrdval: Value=KOUTP_LRWheelTmpHighDTC_raw32_ovrdval
  VDDM_LVSupHiDTC_raw32_Inproc : FVT_lib/outp/OverrideAndLimit  SystemSampleTime=-1  VariantActivationTime=update diagram  Latency=0  AutoFrameSizeCalculation=off
      link override Signal_Limit/_maxval: Value=KOUTP_LVSupHiDTC_raw32_maxval
      link override Signal_Limit/_minval: Value=KOUTP_LVSupHiDTC_raw32_minval
      link override Signal_Override/_ovrdflg: Value=KOUTP_LVSupHiDTC_raw32_ovrdflg
      link override Signal_Override/_ovrdval: Value=KOUTP_LVSupHiDTC_raw32_ovrdval
  VDDM_LVSupLoDTC_raw32_Inproc : FVT_lib/outp/OverrideAndLimit  SystemSampleTime=-1  VariantActivationTime=update diagram  Latency=0  AutoFrameSizeCalculation=off
      link override Signal_Limit/_maxval: Value=KOUTP_LVSupLoDTC_raw32_maxval
      link override Signal_Limit/_minval: Value=KOUTP_LVSupLoDTC_raw32_minval
      link override Signal_Override/_ovrdflg: Value=KOUTP_LVSupLoDTC_raw32_ovrdflg
      link override Signal_Override/_ovrdval: Value=KOUTP_LVSupLoDTC_raw32_ovrdval
  VDDM_LVSysErrPwrOutErr_flg_Inproc : FVT_lib/outp/OverrideAndLimit  SystemSampleTime=-1  VariantActivationTime=update diagram  Latency=0  AutoFrameSizeCalculation=off
      link override Signal_Limit/_maxval: Value=KOUTP_LVSysErrPwrOutErr_flg_maxval
      link override Signal_Limit/_minval: Value=KOUTP_LVSysErrPwrOutErr_flg_minval
      link override Signal_Override/_ovrdflg: Value=KOUTP_LVSysErrPwrOutErr_flg_ovrdflg
      link override Signal_Override/_ovrdval: Value=KOUTP_LVSysErrPwrOutErr_flg_ovrdval
  VDDM_LimpHomeActTmp_flg_Inproc : FVT_lib/outp/OverrideAndLimit  SystemSampleTime=-1  VariantActivationTime=update diagram  Latency=0  AutoFrameSizeCalculation=off
      link override Signal_Limit/_maxval: Value=KOUTP_LimpHomeActTmp_flg_maxval
      link override Signal_Limit/_minval: Value=KOUTP_LimpHomeActTmp_flg_minval
      link override Signal_Override/_ovrdflg: Value=KOUTP_LimpHomeActTmp_flg_ovrdflg
      link override Signal_Override/_ovrdval: Value=KOUTP_LimpHomeActTmp_flg_ovrdval
  VDDM_Lv1ErrDTC_raw32_Inproc : FVT_lib/outp/OverrideAndLimit  SystemSampleTime=-1  VariantActivationTime=update diagram  Latency=0  AutoFrameSizeCalculation=off
      link override Signal_Limit/_maxval: Value=KOUTP_Lv1ErrDTC_raw32_maxval
      link override Signal_Limit/_minval: Value=KOUTP_Lv1ErrDTC_raw32_minval
      link override Signal_Override/_ovrdflg: Value=KOUTP_Lv1ErrDTC_raw32_ovrdflg
      link override Signal_Override/_ovrdval: Value=KOUTP_Lv1ErrDTC_raw32_ovrdval
  VDDM_Lv2ErrDTC_raw32_Inproc : FVT_lib/outp/OverrideAndLimit  SystemSampleTime=-1  VariantActivationTime=update diagram  Latency=0  AutoFrameSizeCalculation=off
      link override Signal_Limit/_maxval: Value=KOUTP_Lv2ErrDTC_raw32_maxval
      link override Signal_Limit/_minval: Value=KOUTP_Lv2ErrDTC_raw32_minval
      link override Signal_Override/_ovrdflg: Value=KOUTP_Lv2ErrDTC_raw32_ovrdflg
      link override Signal_Override/_ovrdval: Value=KOUTP_Lv2ErrDTC_raw32_ovrdval
  VDDM_Lv3ErrDTC_raw32_Inproc : FVT_lib/outp/OverrideAndLimit  SystemSampleTime=-1  VariantActivationTime=update diagram  Latency=0  AutoFrameSizeCalculation=off
      link override Signal_Limit/_maxval: Value=KOUTP_Lv3ErrDTC_raw32_maxval
      link override Signal_Limit/_minval: Value=KOUTP_Lv3ErrDTC_raw32_minval
      link override Signal_Override/_ovrdflg: Value=KOUTP_Lv3ErrDTC_raw32_ovrdflg
      link override Signal_Override/_ovrdval: Value=KOUTP_Lv3ErrDTC_raw32_ovrdval
  VDDM_Lv4ErrDTC_raw32_Inproc : FVT_lib/outp/OverrideAndLimit  SystemSampleTime=-1  VariantActivationTime=update diagram  Latency=0  AutoFrameSizeCalculation=off
      link override Signal_Limit/_maxval: Value=KOUTP_Lv4ErrDTC_raw32_maxval
      link override Signal_Limit/_minval: Value=KOUTP_Lv4ErrDTC_raw32_minval
      link override Signal_Override/_ovrdflg: Value=KOUTP_Lv4ErrDTC_raw32_ovrdflg
      link override Signal_Override/_ovrdval: Value=KOUTP_Lv4ErrDTC_raw32_ovrdval
  VDDM_MCU4PreDTC_raw32_Inproc : FVT_lib/outp/OverrideAndLimit  SystemSampleTime=-1  VariantActivationTime=update diagram  Latency=0  AutoFrameSizeCalculation=off
      link override Signal_Limit/_maxval: Value=KOUTP_MCU4PreDTC_raw32_maxval
      link override Signal_Limit/_minval: Value=KOUTP_MCU4PreDTC_raw32_minval
      link override Signal_Override/_ovrdflg: Value=KOUTP_MCU4PreDTC_raw32_ovrdflg
      link override Signal_Override/_ovrdval: Value=KOUTP_MCU4PreDTC_raw32_ovrdval
  VDDM_MCUActDTC_raw32_Inproc : FVT_lib/outp/OverrideAndLimit  SystemSampleTime=-1  VariantActivationTime=update diagram  Latency=0  AutoFrameSizeCalculation=off
      link override Signal_Limit/_maxval: Value=KOUTP_MCUActDTC_raw32_maxval
      link override Signal_Limit/_minval: Value=KOUTP_MCUActDTC_raw32_minval
      link override Signal_Override/_ovrdflg: Value=KOUTP_MCUActDTC_raw32_ovrdflg
      link override Signal_Override/_ovrdval: Value=KOUTP_MCUActDTC_raw32_ovrdval
  VDDM_MCUActDisFail_flg_Inproc : FVT_lib/outp/OverrideAndLimit  SystemSampleTime=-1  VariantActivationTime=update diagram  Latency=0  AutoFrameSizeCalculation=off
      link override Signal_Limit/_maxval: Value=KOUTP_MCUActDisFail_flg_maxval
      link override Signal_Limit/_minval: Value=KOUTP_MCUActDisFail_flg_minval
      link override Signal_Override/_ovrdflg: Value=KOUTP_MCUActDisFail_flg_ovrdflg
      link override Signal_Override/_ovrdval: Value=KOUTP_MCUActDisFail_flg_ovrdval
  VDDM_MCUDisDTC_raw32_Inproc : FVT_lib/outp/OverrideAndLimit  SystemSampleTime=-1  VariantActivationTime=update diagram  Latency=0  AutoFrameSizeCalculation=off
      link override Signal_Limit/_maxval: Value=KOUTP_MCUDisDTC_raw32_maxval
      link override Signal_Limit/_minval: Value=KOUTP_MCUDisDTC_raw32_minval
      link override Signal_Override/_ovrdflg: Value=KOUTP_MCUDisDTC_raw32_ovrdflg
      link override Signal_Override/_ovrdval: Value=KOUTP_MCUDisDTC_raw32_ovrdval
  VDDM_MCUF1CSErrDTC_raw32_Inproc : FVT_lib/outp/OverrideAndLimit  SystemSampleTime=-1  VariantActivationTime=update diagram  Latency=0  AutoFrameSizeCalculation=off
      link override Signal_Limit/_maxval: Value=KOUTP_MCUF1CSErrDTC_raw32_maxval
      link override Signal_Limit/_minval: Value=KOUTP_MCUF1CSErrDTC_raw32_minval
      link override Signal_Override/_ovrdflg: Value=KOUTP_MCUF1CSErrDTC_raw32_ovrdflg
      link override Signal_Override/_ovrdval: Value=KOUTP_MCUF1CSErrDTC_raw32_ovrdval
  VDDM_MCUF1NoComDTC_raw32_Inproc : FVT_lib/outp/OverrideAndLimit  SystemSampleTime=-1  VariantActivationTime=update diagram  Latency=0  AutoFrameSizeCalculation=off
      link override Signal_Limit/_maxval: Value=KOUTP_MCUF1NoComDTC_raw32_maxval
      link override Signal_Limit/_minval: Value=KOUTP_MCUF1NoComDTC_raw32_minval
      link override Signal_Override/_ovrdflg: Value=KOUTP_MCUF1NoComDTC_raw32_ovrdflg
      link override Signal_Override/_ovrdval: Value=KOUTP_MCUF1NoComDTC_raw32_ovrdval
  VDDM_MCUF1RCErrDTC_raw32_Inproc : FVT_lib/outp/OverrideAndLimit  SystemSampleTime=-1  VariantActivationTime=update diagram  Latency=0  AutoFrameSizeCalculation=off
      link override Signal_Limit/_maxval: Value=KOUTP_MCUF1RCErrDTC_raw32_maxval
      link override Signal_Limit/_minval: Value=KOUTP_MCUF1RCErrDTC_raw32_minval
      link override Signal_Override/_ovrdflg: Value=KOUTP_MCUF1RCErrDTC_raw32_ovrdflg
      link override Signal_Override/_ovrdval: Value=KOUTP_MCUF1RCErrDTC_raw32_ovrdval
  VDDM_MCUR1CSErrDTC_raw32_Inproc : FVT_lib/outp/OverrideAndLimit  SystemSampleTime=-1  VariantActivationTime=update diagram  Latency=0  AutoFrameSizeCalculation=off
      link override Signal_Limit/_maxval: Value=KOUTP_MCUR1CSErrDTC_raw32_maxval
      link override Signal_Limit/_minval: Value=KOUTP_MCUR1CSErrDTC_raw32_minval
      link override Signal_Override/_ovrdflg: Value=KOUTP_MCUR1CSErrDTC_raw32_ovrdflg
      link override Signal_Override/_ovrdval: Value=KOUTP_MCUR1CSErrDTC_raw32_ovrdval
  VDDM_MCUR1NoComDTC_raw32_Inproc : FVT_lib/outp/OverrideAndLimit  SystemSampleTime=-1  VariantActivationTime=update diagram  Latency=0  AutoFrameSizeCalculation=off
      link override Signal_Limit/_maxval: Value=KOUTP_MCUR1NoComDTC_raw32_maxval
      link override Signal_Limit/_minval: Value=KOUTP_MCUR1NoComDTC_raw32_minval
      link override Signal_Override/_ovrdflg: Value=KOUTP_MCUR1NoComDTC_raw32_ovrdflg
      link override Signal_Override/_ovrdval: Value=KOUTP_MCUR1NoComDTC_raw32_ovrdval
  VDDM_MCUR1RCErrDTC_raw32_Inproc : FVT_lib/outp/OverrideAndLimit  SystemSampleTime=-1  VariantActivationTime=update diagram  Latency=0  AutoFrameSizeCalculation=off
      link override Signal_Limit/_maxval: Value=KOUTP_MCUR1RCErrDTC_raw32_maxval
      link override Signal_Limit/_minval: Value=KOUTP_MCUR1RCErrDTC_raw32_minval
      link override Signal_Override/_ovrdflg: Value=KOUTP_MCUR1RCErrDTC_raw32_ovrdflg
      link override Signal_Override/_ovrdval: Value=KOUTP_MCUR1RCErrDTC_raw32_ovrdval
  VDDM_MSAMalfuncDetDTC_raw32_Inproc : FVT_lib/outp/OverrideAndLimit  SystemSampleTime=-1  VariantActivationTime=update diagram  Latency=0  AutoFrameSizeCalculation=off
      link override Signal_Limit/_maxval: Value=KOUTP_MSAMalfuncDetDTC_raw32_maxval
      link override Signal_Limit/_minval: Value=KOUTP_MSAMalfuncDetDTC_raw32_minval
      link override Signal_Override/_ovrdflg: Value=KOUTP_MSAMalfuncDetDTC_raw32_ovrdflg
      link override Signal_Override/_ovrdval: Value=KOUTP_MSAMalfuncDetDTC_raw32_ovrdval
  VDDM_MidLvSaChkDTC_raw32_Inproc : FVT_lib/outp/OverrideAndLimit  SystemSampleTime=-1  VariantActivationTime=update diagram  Latency=0  AutoFrameSizeCalculation=off
      link override Signal_Limit/_maxval: Value=KOUTP_MidLvSaChkDTC_raw32_maxval
      link override Signal_Limit/_minval: Value=KOUTP_MidLvSaChkDTC_raw32_minval
      link override Signal_Override/_ovrdflg: Value=KOUTP_MidLvSaChkDTC_raw32_ovrdflg
      link override Signal_Override/_ovrdval: Value=KOUTP_MidLvSaChkDTC_raw32_ovrdval
  VDDM_OBC4PreDTC_raw32_Inproc : FVT_lib/outp/OverrideAndLimit  SystemSampleTime=-1  VariantActivationTime=update diagram  Latency=0  AutoFrameSizeCalculation=off
      link override Signal_Limit/_maxval: Value=KOUTP_OBC4PreDTC_raw32_maxval
      link override Signal_Limit/_minval: Value=KOUTP_OBC4PreDTC_raw32_minval
      link override Signal_Override/_ovrdflg: Value=KOUTP_OBC4PreDTC_raw32_ovrdflg
      link override Signal_Override/_ovrdval: Value=KOUTP_OBC4PreDTC_raw32_ovrdval
  VDDM_ONtoRdyDTC_raw32_Inproc : FVT_lib/outp/OverrideAndLimit  SystemSampleTime=-1  VariantActivationTime=update diagram  Latency=0  AutoFrameSizeCalculation=off
      link override Signal_Limit/_maxval: Value=KOUTP_ONtoRdyDTC_raw32_maxval
      link override Signal_Limit/_minval: Value=KOUTP_ONtoRdyDTC_raw32_minval
      link override Signal_Override/_ovrdflg: Value=KOUTP_ONtoRdyDTC_raw32_ovrdflg
      link override Signal_Override/_ovrdval: Value=KOUTP_ONtoRdyDTC_raw32_ovrdval
  VDDM_RCLUSSDTC_raw32_Inproc : FVT_lib/outp/OverrideAndLimit  SystemSampleTime=-1  VariantActivationTime=update diagram  Latency=0  AutoFrameSizeCalculation=off
      link override Signal_Limit/_maxval: Value=KOUTP_RCLUSSDTC_raw32_maxval
      link override Signal_Limit/_minval: Value=KOUTP_RCLUSSDTC_raw32_minval
      link override Signal_Override/_ovrdflg: Value=KOUTP_RCLUSSDTC_raw32_ovrdflg
      link override Signal_Override/_ovrdval: Value=KOUTP_RCLUSSDTC_raw32_ovrdval
  VDDM_RCRUSSDTC_raw32_Inproc : FVT_lib/outp/OverrideAndLimit  SystemSampleTime=-1  VariantActivationTime=update diagram  Latency=0  AutoFrameSizeCalculation=off
      link override Signal_Limit/_maxval: Value=KOUTP_RCRUSSDTC_raw32_maxval
      link override Signal_Limit/_minval: Value=KOUTP_RCRUSSDTC_raw32_minval
      link override Signal_Override/_ovrdflg: Value=KOUTP_RCRUSSDTC_raw32_ovrdflg
      link override Signal_Override/_ovrdval: Value=KOUTP_RCRUSSDTC_raw32_ovrdval
  VDDM_RFBatwarnDTC_raw32_Inproc : FVT_lib/outp/OverrideAndLimit  SystemSampleTime=-1  VariantActivationTime=update diagram  Latency=0  AutoFrameSizeCalculation=off
      link override Signal_Limit/_maxval: Value=KOUTP_RFBatwarnDTC_raw32_maxval
      link override Signal_Limit/_minval: Value=KOUTP_RFBatwarnDTC_raw32_minval
      link override Signal_Override/_ovrdflg: Value=KOUTP_RFBatwarnDTC_raw32_ovrdflg
      link override Signal_Override/_ovrdval: Value=KOUTP_RFBatwarnDTC_raw32_ovrdval
  VDDM_RFPressIndiDTC_raw32_Inproc : FVT_lib/outp/OverrideAndLimit  SystemSampleTime=-1  VariantActivationTime=update diagram  Latency=0  AutoFrameSizeCalculation=off
      link override Signal_Limit/_maxval: Value=KOUTP_RFPressIndiDTC_raw32_maxval
      link override Signal_Limit/_minval: Value=KOUTP_RFPressIndiDTC_raw32_minval
      link override Signal_Override/_ovrdflg: Value=KOUTP_RFPressIndiDTC_raw32_ovrdflg
      link override Signal_Override/_ovrdval: Value=KOUTP_RFPressIndiDTC_raw32_ovrdval
  VDDM_RFSensorFailDTC_raw32_Inproc : FVT_lib/outp/OverrideAndLimit  SystemSampleTime=-1  VariantActivationTime=update diagram  Latency=0  AutoFrameSizeCalculation=off
      link override Signal_Limit/_maxval: Value=KOUTP_RFSensorFailDTC_raw32_maxval
      link override Signal_Limit/_minval: Value=KOUTP_RFSensorFailDTC_raw32_minval
      link override Signal_Override/_ovrdflg: Value=KOUTP_RFSensorFailDTC_raw32_ovrdflg
      link override Signal_Override/_ovrdval: Value=KOUTP_RFSensorFailDTC_raw32_ovrdval
  VDDM_RFWheelTmpHighDTC_raw32_Inproc : FVT_lib/outp/OverrideAndLimit  SystemSampleTime=-1  VariantActivationTime=update diagram  Latency=0  AutoFrameSizeCalculation=off
      link override Signal_Limit/_maxval: Value=KOUTP_RFWheelTmpHighDTC_raw32_maxval
      link override Signal_Limit/_minval: Value=KOUTP_RFWheelTmpHighDTC_raw32_minval
      link override Signal_Override/_ovrdflg: Value=KOUTP_RFWheelTmpHighDTC_raw32_ovrdflg
      link override Signal_Override/_ovrdval: Value=KOUTP_RFWheelTmpHighDTC_raw32_ovrdval
  VDDM_RLDoorSWDTC_raw32_Inproc : FVT_lib/outp/OverrideAndLimit  SystemSampleTime=-1  VariantActivationTime=update diagram  Latency=0  AutoFrameSizeCalculation=off
      link override Signal_Limit/_maxval: Value=KOUTP_RLDoorSWDTC_raw32_maxval
      link override Signal_Limit/_minval: Value=KOUTP_RLDoorSWDTC_raw32_minval
      link override Signal_Override/_ovrdflg: Value=KOUTP_RLDoorSWDTC_raw32_ovrdflg
      link override Signal_Override/_ovrdval: Value=KOUTP_RLDoorSWDTC_raw32_ovrdval
  VDDM_RLLUSSDTC_raw32_Inproc : FVT_lib/outp/OverrideAndLimit  SystemSampleTime=-1  VariantActivationTime=update diagram  Latency=0  AutoFrameSizeCalculation=off
      link override Signal_Limit/_maxval: Value=KOUTP_RLLUSSDTC_raw32_maxval
      link override Signal_Limit/_minval: Value=KOUTP_RLLUSSDTC_raw32_minval
      link override Signal_Override/_ovrdflg: Value=KOUTP_RLLUSSDTC_raw32_ovrdflg
      link override Signal_Override/_ovrdval: Value=KOUTP_RLLUSSDTC_raw32_ovrdval
  VDDM_RLRUSSDTC_raw32_Inproc : FVT_lib/outp/OverrideAndLimit  SystemSampleTime=-1  VariantActivationTime=update diagram  Latency=0  AutoFrameSizeCalculation=off
      link override Signal_Limit/_maxval: Value=KOUTP_RLRUSSDTC_raw32_maxval
      link override Signal_Limit/_minval: Value=KOUTP_RLRUSSDTC_raw32_minval
      link override Signal_Override/_ovrdflg: Value=KOUTP_RLRUSSDTC_raw32_ovrdflg
      link override Signal_Override/_ovrdval: Value=KOUTP_RLRUSSDTC_raw32_ovrdval
  VDDM_RMLUSSDTC_raw32_Inproc : FVT_lib/outp/OverrideAndLimit  SystemSampleTime=-1  VariantActivationTime=update diagram  Latency=0  AutoFrameSizeCalculation=off
      link override Signal_Limit/_maxval: Value=KOUTP_RMLUSSDTC_raw32_maxval
      link override Signal_Limit/_minval: Value=KOUTP_RMLUSSDTC_raw32_minval
      link override Signal_Override/_ovrdflg: Value=KOUTP_RMLUSSDTC_raw32_ovrdflg
      link override Signal_Override/_ovrdval: Value=KOUTP_RMLUSSDTC_raw32_ovrdval
  VDDM_RMRUSSDTC_raw32_Inproc : FVT_lib/outp/OverrideAndLimit  SystemSampleTime=-1  VariantActivationTime=update diagram  Latency=0  AutoFrameSizeCalculation=off
      link override Signal_Limit/_maxval: Value=KOUTP_RMRUSSDTC_raw32_maxval
      link override Signal_Limit/_minval: Value=KOUTP_RMRUSSDTC_raw32_minval
      link override Signal_Override/_ovrdflg: Value=KOUTP_RMRUSSDTC_raw32_ovrdflg
      link override Signal_Override/_ovrdval: Value=KOUTP_RMRUSSDTC_raw32_ovrdval
  VDDM_RRBatwarnDTC_raw32_Inproc : FVT_lib/outp/OverrideAndLimit  SystemSampleTime=-1  VariantActivationTime=update diagram  Latency=0  AutoFrameSizeCalculation=off
      link override Signal_Limit/_maxval: Value=KOUTP_RRBatwarnDTC_raw32_maxval
      link override Signal_Limit/_minval: Value=KOUTP_RRBatwarnDTC_raw32_minval
      link override Signal_Override/_ovrdflg: Value=KOUTP_RRBatwarnDTC_raw32_ovrdflg
      link override Signal_Override/_ovrdval: Value=KOUTP_RRBatwarnDTC_raw32_ovrdval
  VDDM_RRDoorSWDTC_raw32_Inproc : FVT_lib/outp/OverrideAndLimit  SystemSampleTime=-1  VariantActivationTime=update diagram  Latency=0  AutoFrameSizeCalculation=off
      link override Signal_Limit/_maxval: Value=KOUTP_RRDoorSWDTC_raw32_maxval
      link override Signal_Limit/_minval: Value=KOUTP_RRDoorSWDTC_raw32_minval
      link override Signal_Override/_ovrdflg: Value=KOUTP_RRDoorSWDTC_raw32_ovrdflg
      link override Signal_Override/_ovrdval: Value=KOUTP_RRDoorSWDTC_raw32_ovrdval
  VDDM_RRPressIndiDTC_raw32_Inproc : FVT_lib/outp/OverrideAndLimit  SystemSampleTime=-1  VariantActivationTime=update diagram  Latency=0  AutoFrameSizeCalculation=off
      link override Signal_Limit/_maxval: Value=KOUTP_RRPressIndiDTC_raw32_maxval
      link override Signal_Limit/_minval: Value=KOUTP_RRPressIndiDTC_raw32_minval
      link override Signal_Override/_ovrdflg: Value=KOUTP_RRPressIndiDTC_raw32_ovrdflg
      link override Signal_Override/_ovrdval: Value=KOUTP_RRPressIndiDTC_raw32_ovrdval
  VDDM_RRSensorFailDTC_raw32_Inproc : FVT_lib/outp/OverrideAndLimit  SystemSampleTime=-1  VariantActivationTime=update diagram  Latency=0  AutoFrameSizeCalculation=off
      link override Signal_Limit/_maxval: Value=KOUTP_RRSensorFailDTC_raw32_maxval
      link override Signal_Limit/_minval: Value=KOUTP_RRSensorFailDTC_raw32_minval
      link override Signal_Override/_ovrdflg: Value=KOUTP_RRSensorFailDTC_raw32_ovrdflg
      link override Signal_Override/_ovrdval: Value=KOUTP_RRSensorFailDTC_raw32_ovrdval
  VDDM_RRWheelTmpHighDTC_raw32_Inproc : FVT_lib/outp/OverrideAndLimit  SystemSampleTime=-1  VariantActivationTime=update diagram  Latency=0  AutoFrameSizeCalculation=off
      link override Signal_Limit/_maxval: Value=KOUTP_RRWheelTmpHighDTC_raw32_maxval
      link override Signal_Limit/_minval: Value=KOUTP_RRWheelTmpHighDTC_raw32_minval
      link override Signal_Override/_ovrdflg: Value=KOUTP_RRWheelTmpHighDTC_raw32_ovrdflg
      link override Signal_Override/_ovrdval: Value=KOUTP_RRWheelTmpHighDTC_raw32_ovrdval
  VDDM_RrMCUSigErrDetDTC_raw32_Inproc : FVT_lib/outp/OverrideAndLimit  SystemSampleTime=-1  VariantActivationTime=update diagram  Latency=0  AutoFrameSizeCalculation=off
      link override Signal_Limit/_maxval: Value=KOUTP_RrMCUSigErrDetDTC_raw32_maxval
      link override Signal_Limit/_minval: Value=KOUTP_RrMCUSigErrDetDTC_raw32_minval
      link override Signal_Override/_ovrdflg: Value=KOUTP_RrMCUSigErrDetDTC_raw32_ovrdflg
      link override Signal_Override/_ovrdval: Value=KOUTP_RrMCUSigErrDetDTC_raw32_ovrdval
  VDDM_RrMCUTqErrDTC_raw32_Inproc : FVT_lib/outp/OverrideAndLimit  SystemSampleTime=-1  VariantActivationTime=update diagram  Latency=0  AutoFrameSizeCalculation=off
      link override Signal_Limit/_maxval: Value=KOUTP_RrMCUTqErrDTC_raw32_maxval
      link override Signal_Limit/_minval: Value=KOUTP_RrMCUTqErrDTC_raw32_minval
      link override Signal_Override/_ovrdflg: Value=KOUTP_RrMCUTqErrDTC_raw32_ovrdflg
      link override Signal_Override/_ovrdval: Value=KOUTP_RrMCUTqErrDTC_raw32_ovrdval
  VDDM_Shifter1CSErrDTC_raw32_Inproc : FVT_lib/outp/OverrideAndLimit  SystemSampleTime=-1  VariantActivationTime=update diagram  Latency=0  AutoFrameSizeCalculation=off
      link override Signal_Limit/_maxval: Value=KOUTP_Shifter1CSErrDTC_raw32_maxval
      link override Signal_Limit/_minval: Value=KOUTP_Shifter1CSErrDTC_raw32_minval
      link override Signal_Override/_ovrdflg: Value=KOUTP_Shifter1CSErrDTC_raw32_ovrdflg
      link override Signal_Override/_ovrdval: Value=KOUTP_Shifter1CSErrDTC_raw32_ovrdval
  VDDM_Shifter1NoComDTC_raw32_Inproc : FVT_lib/outp/OverrideAndLimit  SystemSampleTime=-1  VariantActivationTime=update diagram  Latency=0  AutoFrameSizeCalculation=off
      link override Signal_Limit/_maxval: Value=KOUTP_Shifter1NoComDTC_raw32_maxval
      link override Signal_Limit/_minval: Value=KOUTP_Shifter1NoComDTC_raw32_minval
      link override Signal_Override/_ovrdflg: Value=KOUTP_Shifter1NoComDTC_raw32_ovrdflg
      link override Signal_Override/_ovrdval: Value=KOUTP_Shifter1NoComDTC_raw32_ovrdval
  VDDM_Shifter1RCErrDTC_raw32_Inproc : FVT_lib/outp/OverrideAndLimit  SystemSampleTime=-1  VariantActivationTime=update diagram  Latency=0  AutoFrameSizeCalculation=off
      link override Signal_Limit/_maxval: Value=KOUTP_Shifter1RCErrDTC_raw32_maxval
      link override Signal_Limit/_minval: Value=KOUTP_Shifter1RCErrDTC_raw32_minval
      link override Signal_Override/_ovrdflg: Value=KOUTP_Shifter1RCErrDTC_raw32_ovrdflg
      link override Signal_Override/_ovrdval: Value=KOUTP_Shifter1RCErrDTC_raw32_ovrdval
  VDDM_SysAllowReadySta_flg_Inproc : FVT_lib/outp/OverrideAndLimit  SystemSampleTime=-1  VariantActivationTime=update diagram  Latency=0  AutoFrameSizeCalculation=off
      link override Signal_Limit/_maxval: Value=KOUTP_SysAllowReadySta_flg_maxval
      link override Signal_Limit/_minval: Value=KOUTP_SysAllowReadySta_flg_minval
      link override Signal_Override/_ovrdflg: Value=KOUTP_SysAllowReadySta_flg_ovrdflg
      link override Signal_Override/_ovrdval: Value=KOUTP_SysAllowReadySta_flg_ovrdval
  VDDM_TailgaSWDTC_raw32_Inproc : FVT_lib/outp/OverrideAndLimit  SystemSampleTime=-1  VariantActivationTime=update diagram  Latency=0  AutoFrameSizeCalculation=off
      link override Signal_Limit/_maxval: Value=KOUTP_TailgaSWDTC_raw32_maxval
      link override Signal_Limit/_minval: Value=KOUTP_TailgaSWDTC_raw32_minval
      link override Signal_Override/_ovrdflg: Value=KOUTP_TailgaSWDTC_raw32_ovrdflg
      link override Signal_Override/_ovrdval: Value=KOUTP_TailgaSWDTC_raw32_ovrdval
  VDDM_VCUBrkSWSta_enum_Inproc : FVT_lib/outp/OverrideAndLimit  SystemSampleTime=-1  VariantActivationTime=update diagram  Latency=0  AutoFrameSizeCalculation=off
      link override Signal_Limit/_maxval: Value=KOUTP_VCUBrkSWSta_enum_maxval
      link override Signal_Limit/_minval: Value=KOUTP_VCUBrkSWSta_enum_minval
      link override Signal_Override/_ovrdflg: Value=KOUTP_VCUBrkSWSta_enum_ovrdflg
      link override Signal_Override/_ovrdval: Value=KOUTP_VCUBrkSWSta_enum_ovrdval
  VDDM_VCUFLDoorSta_flg_Inproc : FVT_lib/outp/OverrideAndLimit  SystemSampleTime=-1  VariantActivationTime=update diagram  Latency=0  AutoFrameSizeCalculation=off
      link override Signal_Limit/_maxval: Value=KOUTP_VCUFLDoorSta_flg_maxval
      link override Signal_Limit/_minval: Value=KOUTP_VCUFLDoorSta_flg_minval
      link override Signal_Override/_ovrdflg: Value=KOUTP_VCUFLDoorSta_flg_ovrdflg
      link override Signal_Override/_ovrdval: Value=KOUTP_VCUFLDoorSta_flg_ovrdval
  VDDM_VCUFRDoorSta_flg_Inproc : FVT_lib/outp/OverrideAndLimit  SystemSampleTime=-1  VariantActivationTime=update diagram  Latency=0  AutoFrameSizeCalculation=off
      link override Signal_Limit/_maxval: Value=KOUTP_VCUFRDoorSta_flg_maxval
      link override Signal_Limit/_minval: Value=KOUTP_VCUFRDoorSta_flg_minval
      link override Signal_Override/_ovrdflg: Value=KOUTP_VCUFRDoorSta_flg_ovrdflg
      link override Signal_Override/_ovrdval: Value=KOUTP_VCUFRDoorSta_flg_ovrdval
  VDDM_VCUHoodSWSta_flg_Inproc : FVT_lib/outp/OverrideAndLimit  SystemSampleTime=-1  VariantActivationTime=update diagram  Latency=0  AutoFrameSizeCalculation=off
      link override Signal_Limit/_maxval: Value=KOUTP_VCUHoodSWSta_flg_maxval
      link override Signal_Limit/_minval: Value=KOUTP_VCUHoodSWSta_flg_minval
      link override Signal_Override/_ovrdflg: Value=KOUTP_VCUHoodSWSta_flg_ovrdflg
      link override Signal_Override/_ovrdval: Value=KOUTP_VCUHoodSWSta_flg_ovrdval
  VDDM_VCURAPSErrLv2_flg_Inproc : FVT_lib/outp/OverrideAndLimit  SystemSampleTime=-1  VariantActivationTime=update diagram  Latency=0  AutoFrameSizeCalculation=off
      link override Signal_Limit/_maxval: Value=KOUTP_VCURAPSErrLv2_flg_maxval
      link override Signal_Limit/_minval: Value=KOUTP_VCURAPSErrLv2_flg_minval
      link override Signal_Override/_ovrdflg: Value=KOUTP_VCURAPSErrLv2_flg_ovrdflg
      link override Signal_Override/_ovrdval: Value=KOUTP_VCURAPSErrLv2_flg_ovrdval
  VDDM_VCURAPSErrLv3_flg_Inproc : FVT_lib/outp/OverrideAndLimit  SystemSampleTime=-1  VariantActivationTime=update diagram  Latency=0  AutoFrameSizeCalculation=off
      link override Signal_Limit/_maxval: Value=KOUTP_VCURAPSErrLv3_flg_maxval
      link override Signal_Limit/_minval: Value=KOUTP_VCURAPSErrLv3_flg_minval
      link override Signal_Override/_ovrdflg: Value=KOUTP_VCURAPSErrLv3_flg_ovrdflg
      link override Signal_Override/_ovrdval: Value=KOUTP_VCURAPSErrLv3_flg_ovrdval
  VDDM_VCURLDoorSta_flg_Inproc : FVT_lib/outp/OverrideAndLimit  SystemSampleTime=-1  VariantActivationTime=update diagram  Latency=0  AutoFrameSizeCalculation=off
      link override Signal_Limit/_maxval: Value=KOUTP_VCURLDoorSta_flg_maxval
      link override Signal_Limit/_minval: Value=KOUTP_VCURLDoorSta_flg_minval
      link override Signal_Override/_ovrdflg: Value=KOUTP_VCURLDoorSta_flg_ovrdflg
      link override Signal_Override/_ovrdval: Value=KOUTP_VCURLDoorSta_flg_ovrdval
  VDDM_VCURRDoorSta_flg_Inproc : FVT_lib/outp/OverrideAndLimit  SystemSampleTime=-1  VariantActivationTime=update diagram  Latency=0  AutoFrameSizeCalculation=off
      link override Signal_Limit/_maxval: Value=KOUTP_VCURRDoorSta_flg_maxval
      link override Signal_Limit/_minval: Value=KOUTP_VCURRDoorSta_flg_minval
      link override Signal_Override/_ovrdflg: Value=KOUTP_VCURRDoorSta_flg_ovrdflg
      link override Signal_Override/_ovrdval: Value=KOUTP_VCURRDoorSta_flg_ovrdval
  VDDM_VCUTailgateSWSta_flg_Inproc : FVT_lib/outp/OverrideAndLimit  SystemSampleTime=-1  VariantActivationTime=update diagram  Latency=0  AutoFrameSizeCalculation=off
      link override Signal_Limit/_maxval: Value=KOUTP_VCUTailgateSWSta_flg_maxval
      link override Signal_Limit/_minval: Value=KOUTP_VCUTailgateSWSta_flg_minval
      link override Signal_Override/_ovrdflg: Value=KOUTP_VCUTailgateSWSta_flg_ovrdflg
      link override Signal_Override/_ovrdval: Value=KOUTP_VCUTailgateSWSta_flg_ovrdval
  VDDM_VehMalfunLevel_enum_Inproc : FVT_lib/outp/OverrideAndLimit  SystemSampleTime=-1  VariantActivationTime=update diagram  Latency=0  AutoFrameSizeCalculation=off
      link override Signal_Limit/_maxval: Value=KOUTP_VehMalfunLevel_enum_maxval
      link override Signal_Limit/_minval: Value=KOUTP_VehMalfunLevel_enum_minval
      link override Signal_Override/_ovrdflg: Value=KOUTP_VehMalfunLevel_enum_ovrdflg
      link override Signal_Override/_ovrdval: Value=KOUTP_VehMalfunLevel_enum_ovrdval
  VDDM_ZoneSCPNoComDTC_raw32_Inproc : FVT_lib/outp/OverrideAndLimit  SystemSampleTime=-1  VariantActivationTime=update diagram  Latency=0  AutoFrameSizeCalculation=off
      link override Signal_Limit/_maxval: Value=KOUTP_ZoneSCPNoComDTC_raw32_maxval
      link override Signal_Limit/_minval: Value=KOUTP_ZoneSCPNoComDTC_raw32_minval
      link override Signal_Override/_ovrdflg: Value=KOUTP_ZoneSCPNoComDTC_raw32_ovrdflg
      link override Signal_Override/_ovrdval: Value=KOUTP_ZoneSCPNoComDTC_raw32_ovrdval
  VDHP_ActAPSPosn_pct_Inproc : FVT_lib/outp/OverrideAndLimit  SystemSampleTime=-1  VariantActivationTime=update diagram  Latency=0  AutoFrameSizeCalculation=off
      link override Signal_Limit/_maxval: Value=KOUTP_ActAPSPosn_pct_maxval
      link override Signal_Limit/_minval: Value=KOUTP_ActAPSPosn_pct_minval
      link override Signal_Override/_ovrdflg: Value=KOUTP_ActAPSPosn_pct_ovrdflg
      link override Signal_Override/_ovrdval: Value=KOUTP_ActAPSPosn_pct_ovrdval
  VDHP_EAPS1MIN_pct_Inproc : FVT_lib/outp/OverrideAndLimit  SystemSampleTime=-1  VariantActivationTime=update diagram  Latency=0  AutoFrameSizeCalculation=off
      link override Signal_Limit/_maxval: Value=KOUTP_EAPS1MIN_pct_maxval
      link override Signal_Limit/_minval: Value=KOUTP_EAPS1MIN_pct_minval
      link override Signal_Override/_ovrdflg: Value=KOUTP_EAPS1MIN_pct_ovrdflg
      link override Signal_Override/_ovrdval: Value=KOUTP_EAPS1MIN_pct_ovrdval
  VDHP_EAPS1NRM_pct_Inproc : FVT_lib/outp/OverrideAndLimit  SystemSampleTime=-1  VariantActivationTime=update diagram  Latency=0  AutoFrameSizeCalculation=off
      link override Signal_Limit/_maxval: Value=KOUTP_EAPS1NRM_pct_maxval
      link override Signal_Limit/_minval: Value=KOUTP_EAPS1NRM_pct_minval
      link override Signal_Override/_ovrdflg: Value=KOUTP_EAPS1NRM_pct_ovrdflg
      link override Signal_Override/_ovrdval: Value=KOUTP_EAPS1NRM_pct_ovrdval
  VDHP_EAPS2MIN_pct_Inproc : FVT_lib/outp/OverrideAndLimit  SystemSampleTime=-1  VariantActivationTime=update diagram  Latency=0  AutoFrameSizeCalculation=off
      link override Signal_Limit/_maxval: Value=KOUTP_EAPS2MIN_pct_maxval
      link override Signal_Limit/_minval: Value=KOUTP_EAPS2MIN_pct_minval
      link override Signal_Override/_ovrdflg: Value=KOUTP_EAPS2MIN_pct_ovrdflg
      link override Signal_Override/_ovrdval: Value=KOUTP_EAPS2MIN_pct_ovrdval
  VDHP_EAPS2NRM_pct_Inproc : FVT_lib/outp/OverrideAndLimit  SystemSampleTime=-1  VariantActivationTime=update diagram  Latency=0  AutoFrameSizeCalculation=off
      link override Signal_Limit/_maxval: Value=KOUTP_EAPS2NRM_pct_maxval
      link override Signal_Limit/_minval: Value=KOUTP_EAPS2NRM_pct_minval
      link override Signal_Override/_ovrdflg: Value=KOUTP_EAPS2NRM_pct_ovrdflg
      link override Signal_Override/_ovrdval: Value=KOUTP_EAPS2NRM_pct_ovrdval
  VDHP_ResetPedalZeroPosStart_flg_Inproc : FVT_lib/outp/OverrideAndLimit  SystemSampleTime=-1  VariantActivationTime=update diagram  Latency=0  AutoFrameSizeCalculation=off
      link override Signal_Limit/_maxval: Value=KOUTP_ResetPedalZeroPosStart_flg_maxval
      link override Signal_Limit/_minval: Value=KOUTP_ResetPedalZeroPosStart_flg_minval
      link override Signal_Override/_ovrdflg: Value=KOUTP_ResetPedalZeroPosStart_flg_ovrdflg
      link override Signal_Override/_ovrdval: Value=KOUTP_ResetPedalZeroPosStart_flg_ovrdval
  VDID_APPD_pct_Inproc : FVT_lib/outp/OverrideAndLimit  SystemSampleTime=-1  VariantActivationTime=update diagram  Latency=0  AutoFrameSizeCalculation=off
      link override Signal_Limit/_maxval: Value=KOUTP_APPD_pct_maxval
      link override Signal_Limit/_minval: Value=KOUTP_APPD_pct_minval
      link override Signal_Override/_ovrdflg: Value=KOUTP_APPD_pct_ovrdflg
      link override Signal_Override/_ovrdval: Value=KOUTP_APPD_pct_ovrdval
  VDID_APPE_pct_Inproc : FVT_lib/outp/OverrideAndLimit  SystemSampleTime=-1  VariantActivationTime=update diagram  Latency=0  AutoFrameSizeCalculation=off
      link override Signal_Limit/_maxval: Value=KOUTP_APPE_pct_maxval
      link override Signal_Limit/_minval: Value=KOUTP_APPE_pct_minval
      link override Signal_Override/_ovrdflg: Value=KOUTP_APPE_pct_ovrdflg
      link override Signal_Override/_ovrdval: Value=KOUTP_APPE_pct_ovrdval
  VDID_AVGBATTEMPL_C_Inproc : FVT_lib/outp/OverrideAndLimit  SystemSampleTime=-1  VariantActivationTime=update diagram  Latency=0  AutoFrameSizeCalculation=off
      link override Signal_Limit/_maxval: Value=KOUTP_AVGBATTEMPL_C_maxval
      link override Signal_Limit/_minval: Value=KOUTP_AVGBATTEMPL_C_minval
      link override Signal_Override/_ovrdflg: Value=KOUTP_AVGBATTEMPL_C_ovrdflg
      link override Signal_Override/_ovrdval: Value=KOUTP_AVGBATTEMPL_C_ovrdval
  VDID_AVGBATTEMPL_sec_Inproc : FVT_lib/outp/OverrideAndLimit  SystemSampleTime=-1  VariantActivationTime=update diagram  Latency=0  AutoFrameSizeCalculation=off
      link override Signal_Limit/_maxval: Value=KOUTP_AVGBATTEMPL_sec_maxval
      link override Signal_Limit/_minval: Value=KOUTP_AVGBATTEMPL_sec_minval
      link override Signal_Override/_ovrdflg: Value=KOUTP_AVGBATTEMPL_sec_ovrdflg
      link override Signal_Override/_ovrdval: Value=KOUTP_AVGBATTEMPL_sec_ovrdval
  VDID_AvgBattTempOFFL_C_Inproc : FVT_lib/outp/OverrideAndLimit  SystemSampleTime=-1  VariantActivationTime=update diagram  Latency=0  AutoFrameSizeCalculation=off
      link override Signal_Limit/_maxval: Value=KOUTP_AvgBattTempOFFL_C_maxval
      link override Signal_Limit/_minval: Value=KOUTP_AvgBattTempOFFL_C_minval
      link override Signal_Override/_ovrdflg: Value=KOUTP_AvgBattTempOFFL_C_ovrdflg
      link override Signal_Override/_ovrdval: Value=KOUTP_AvgBattTempOFFL_C_ovrdval
  VDID_AvgBattTempOFFR_C_Inproc : FVT_lib/outp/OverrideAndLimit  SystemSampleTime=-1  VariantActivationTime=update diagram  Latency=0  AutoFrameSizeCalculation=off
      link override Signal_Limit/_maxval: Value=KOUTP_AvgBattTempOFFR_C_maxval
      link override Signal_Limit/_minval: Value=KOUTP_AvgBattTempOFFR_C_minval
      link override Signal_Override/_ovrdflg: Value=KOUTP_AvgBattTempOFFR_C_ovrdflg
      link override Signal_Override/_ovrdval: Value=KOUTP_AvgBattTempOFFR_C_ovrdval
  VDID_AvgBattTempOVCL_C_Inproc : FVT_lib/outp/OverrideAndLimit  SystemSampleTime=-1  VariantActivationTime=update diagram  Latency=0  AutoFrameSizeCalculation=off
      link override Signal_Limit/_maxval: Value=KOUTP_AvgBattTempOVCL_C_maxval
      link override Signal_Limit/_minval: Value=KOUTP_AvgBattTempOVCL_C_minval
      link override Signal_Override/_ovrdflg: Value=KOUTP_AvgBattTempOVCL_C_ovrdflg
      link override Signal_Override/_ovrdval: Value=KOUTP_AvgBattTempOVCL_C_ovrdval
  VDID_AvgBattTempOVCR_C_Inproc : FVT_lib/outp/OverrideAndLimit  SystemSampleTime=-1  VariantActivationTime=update diagram  Latency=0  AutoFrameSizeCalculation=off
      link override Signal_Limit/_maxval: Value=KOUTP_AvgBattTempOVCR_C_maxval
      link override Signal_Limit/_minval: Value=KOUTP_AvgBattTempOVCR_C_minval
      link override Signal_Override/_ovrdflg: Value=KOUTP_AvgBattTempOVCR_C_ovrdflg
      link override Signal_Override/_ovrdval: Value=KOUTP_AvgBattTempOVCR_C_ovrdval
  VDID_AvgBattTempPSAL_C_Inproc : FVT_lib/outp/OverrideAndLimit  SystemSampleTime=-1  VariantActivationTime=update diagram  Latency=0  AutoFrameSizeCalculation=off
      link override Signal_Limit/_maxval: Value=KOUTP_AvgBattTempPSAL_C_maxval
      link override Signal_Limit/_minval: Value=KOUTP_AvgBattTempPSAL_C_minval
      link override Signal_Override/_ovrdflg: Value=KOUTP_AvgBattTempPSAL_C_ovrdflg
      link override Signal_Override/_ovrdval: Value=KOUTP_AvgBattTempPSAL_C_ovrdval
  VDID_AvgBattTempPSAR_C_Inproc : FVT_lib/outp/OverrideAndLimit  SystemSampleTime=-1  VariantActivationTime=update diagram  Latency=0  AutoFrameSizeCalculation=off
      link override Signal_Limit/_maxval: Value=KOUTP_AvgBattTempPSAR_C_maxval
      link override Signal_Limit/_minval: Value=KOUTP_AvgBattTempPSAR_C_minval
      link override Signal_Override/_ovrdflg: Value=KOUTP_AvgBattTempPSAR_C_ovrdflg
      link override Signal_Override/_ovrdval: Value=KOUTP_AvgBattTempPSAR_C_ovrdval
  VDID_BATSOC_pct_Inproc : FVT_lib/outp/OverrideAndLimit  SystemSampleTime=-1  VariantActivationTime=update diagram  Latency=0  AutoFrameSizeCalculation=off
      link override Signal_Limit/_maxval: Value=KOUTP_BATSOC_pct_maxval
      link override Signal_Limit/_minval: Value=KOUTP_BATSOC_pct_minval
      link override Signal_Override/_ovrdflg: Value=KOUTP_BATSOC_pct_ovrdflg
      link override Signal_Override/_ovrdval: Value=KOUTP_BATSOC_pct_ovrdval
  VDID_BATSOH_pct_Inproc : FVT_lib/outp/OverrideAndLimit  SystemSampleTime=-1  VariantActivationTime=update diagram  Latency=0  AutoFrameSizeCalculation=off
      link override Signal_Limit/_maxval: Value=KOUTP_BATSOH_pct_maxval
      link override Signal_Limit/_minval: Value=KOUTP_BATSOH_pct_minval
      link override Signal_Override/_ovrdflg: Value=KOUTP_BATSOH_pct_ovrdflg
      link override Signal_Override/_ovrdval: Value=KOUTP_BATSOH_pct_ovrdval
  VDID_BattTempPSAL_sec_Inproc : FVT_lib/outp/OverrideAndLimit  SystemSampleTime=-1  VariantActivationTime=update diagram  Latency=0  AutoFrameSizeCalculation=off
      link override Signal_Limit/_maxval: Value=KOUTP_BattTempPSAL_sec_maxval
      link override Signal_Limit/_minval: Value=KOUTP_BattTempPSAL_sec_minval
      link override Signal_Override/_ovrdflg: Value=KOUTP_BattTempPSAL_sec_ovrdflg
      link override Signal_Override/_ovrdval: Value=KOUTP_BattTempPSAL_sec_ovrdval
  VDID_BattTempPSAR_sec_Inproc : FVT_lib/outp/OverrideAndLimit  SystemSampleTime=-1  VariantActivationTime=update diagram  Latency=0  AutoFrameSizeCalculation=off
      link override Signal_Limit/_maxval: Value=KOUTP_BattTempPSAR_sec_maxval
      link override Signal_Limit/_minval: Value=KOUTP_BattTempPSAR_sec_minval
      link override Signal_Override/_ovrdflg: Value=KOUTP_BattTempPSAR_sec_ovrdflg
      link override Signal_Override/_ovrdval: Value=KOUTP_BattTempPSAR_sec_ovrdval
  VDID_CALID_cnt_Inproc : FVT_lib/outp/OverrideAndLimit  SystemSampleTime=-1  VariantActivationTime=update diagram  Latency=0  AutoFrameSizeCalculation=off
      link override Signal_Limit/_maxval: Value=KOUTP_CALID_cnt_maxval
      link override Signal_Limit/_minval: Value=KOUTP_CALID_cnt_minval
      link override Signal_Override/_ovrdflg: Value=KOUTP_CALID_cnt_ovrdflg
      link override Signal_Override/_ovrdval: Value=KOUTP_CALID_cnt_ovrdval
  VDID_CDEODTL_km_Inproc : FVT_lib/outp/OverrideAndLimit  SystemSampleTime=-1  VariantActivationTime=update diagram  Latency=0  AutoFrameSizeCalculation=off
      link override Signal_Limit/_maxval: Value=KOUTP_CDEODTL_km_maxval
      link override Signal_Limit/_minval: Value=KOUTP_CDEODTL_km_minval
      link override Signal_Override/_ovrdflg: Value=KOUTP_CDEODTL_km_ovrdflg
      link override Signal_Override/_ovrdval: Value=KOUTP_CDEODTL_km_ovrdval
  VDID_CDEODTR_km_Inproc : FVT_lib/outp/OverrideAndLimit  SystemSampleTime=-1  VariantActivationTime=update diagram  Latency=0  AutoFrameSizeCalculation=off
      link override Signal_Limit/_maxval: Value=KOUTP_CDEODTR_km_maxval
      link override Signal_Limit/_minval: Value=KOUTP_CDEODTR_km_minval
      link override Signal_Override/_ovrdflg: Value=KOUTP_CDEODTR_km_ovrdflg
      link override Signal_Override/_ovrdval: Value=KOUTP_CDEODTR_km_ovrdval
  VDID_CLRDIST_km_Inproc : FVT_lib/outp/OverrideAndLimit  SystemSampleTime=-1  VariantActivationTime=update diagram  Latency=0  AutoFrameSizeCalculation=off
      link override Signal_Limit/_maxval: Value=KOUTP_CLRDIST_km_maxval
      link override Signal_Limit/_minval: Value=KOUTP_CLRDIST_km_minval
      link override Signal_Override/_ovrdflg: Value=KOUTP_CLRDIST_km_ovrdflg
      link override Signal_Override/_ovrdval: Value=KOUTP_CLRDIST_km_ovrdval
  VDID_CLRTIME_min_Inproc : FVT_lib/outp/OverrideAndLimit  SystemSampleTime=-1  VariantActivationTime=update diagram  Latency=0  AutoFrameSizeCalculation=off
      link override Signal_Limit/_maxval: Value=KOUTP_CLRTIME_min_maxval
      link override Signal_Limit/_minval: Value=KOUTP_CLRTIME_min_minval
      link override Signal_Override/_ovrdflg: Value=KOUTP_CLRTIME_min_ovrdflg
      link override Signal_Override/_ovrdval: Value=KOUTP_CLRTIME_min_ovrdval
  VDID_CPSAL_sec_Inproc : FVT_lib/outp/OverrideAndLimit  SystemSampleTime=-1  VariantActivationTime=update diagram  Latency=0  AutoFrameSizeCalculation=off
      link override Signal_Limit/_maxval: Value=KOUTP_CPSAL_sec_maxval
      link override Signal_Limit/_minval: Value=KOUTP_CPSAL_sec_minval
      link override Signal_Override/_ovrdflg: Value=KOUTP_CPSAL_sec_ovrdflg
      link override Signal_Override/_ovrdval: Value=KOUTP_CPSAL_sec_ovrdval
  VDID_CPSAR_sec_Inproc : FVT_lib/outp/OverrideAndLimit  SystemSampleTime=-1  VariantActivationTime=update diagram  Latency=0  AutoFrameSizeCalculation=off
      link override Signal_Limit/_maxval: Value=KOUTP_CPSAR_sec_maxval
      link override Signal_Limit/_minval: Value=KOUTP_CPSAR_sec_minval
      link override Signal_Override/_ovrdflg: Value=KOUTP_CPSAR_sec_ovrdflg
      link override Signal_Override/_ovrdval: Value=KOUTP_CPSAR_sec_ovrdval
  VDID_DIDModelVersionChksum_raw_Inproc : FVT_lib/outp/OverrideAndLimit  SystemSampleTime=-1  VariantActivationTime=update diagram  Latency=0  AutoFrameSizeCalculation=off
      link override Signal_Limit/_maxval: Value=KOUTP_DIDModelVersionChksum_raw_maxval
      link override Signal_Limit/_minval: Value=KOUTP_DIDModelVersionChksum_raw_minval
      link override Signal_Override/_ovrdflg: Value=KOUTP_DIDModelVersionChksum_raw_ovrdflg
      link override Signal_Override/_ovrdval: Value=KOUTP_DIDModelVersionChksum_raw_ovrdval
  VDID_DIDModelVersion_raw_Inproc : FVT_lib/outp/OverrideAndLimit  SystemSampleTime=-1  VariantActivationTime=update diagram  Latency=0  AutoFrameSizeCalculation=off
      link override Signal_Limit/_maxval: Value=KOUTP_DIDModelVersion_raw_maxval
      link override Signal_Limit/_minval: Value=KOUTP_DIDModelVersion_raw_minval
      link override Signal_Override/_ovrdflg: Value=KOUTP_DIDModelVersion_raw_ovrdflg
      link override Signal_Override/_ovrdval: Value=KOUTP_DIDModelVersion_raw_ovrdval
  VDID_ECUNAME_cnt_Inproc : FVT_lib/outp/OverrideAndLimit  SystemSampleTime=-1  VariantActivationTime=update diagram  Latency=0  AutoFrameSizeCalculation=off
      link override Signal_Limit/_maxval: Value=KOUTP_ECUNAME_cnt_maxval
      link override Signal_Limit/_minval: Value=KOUTP_ECUNAME_cnt_minval
      link override Signal_Override/_ovrdflg: Value=KOUTP_ECUNAME_cnt_ovrdflg
      link override Signal_Override/_ovrdval: Value=KOUTP_ECUNAME_cnt_ovrdval
  VDID_ETMATOEL_kWh_Inproc : FVT_lib/outp/OverrideAndLimit  SystemSampleTime=-1  VariantActivationTime=update diagram  Latency=0  AutoFrameSizeCalculation=off
      link override Signal_Limit/_maxval: Value=KOUTP_ETMATOEL_kWh_maxval
      link override Signal_Limit/_minval: Value=KOUTP_ETMATOEL_kWh_minval
      link override Signal_Override/_ovrdflg: Value=KOUTP_ETMATOEL_kWh_ovrdflg
      link override Signal_Override/_ovrdval: Value=KOUTP_ETMATOEL_kWh_ovrdval
  VDID_ETMATOER_kWh_Inproc : FVT_lib/outp/OverrideAndLimit  SystemSampleTime=-1  VariantActivationTime=update diagram  Latency=0  AutoFrameSizeCalculation=off
      link override Signal_Limit/_maxval: Value=KOUTP_ETMATOER_kWh_maxval
      link override Signal_Limit/_minval: Value=KOUTP_ETMATOER_kWh_minval
      link override Signal_Override/_ovrdflg: Value=KOUTP_ETMATOER_kWh_ovrdflg
      link override Signal_Override/_ovrdval: Value=KOUTP_ETMATOER_kWh_ovrdval
  VDID_ETMBTOEL_kWh_Inproc : FVT_lib/outp/OverrideAndLimit  SystemSampleTime=-1  VariantActivationTime=update diagram  Latency=0  AutoFrameSizeCalculation=off
      link override Signal_Limit/_maxval: Value=KOUTP_ETMBTOEL_kWh_maxval
      link override Signal_Limit/_minval: Value=KOUTP_ETMBTOEL_kWh_minval
      link override Signal_Override/_ovrdflg: Value=KOUTP_ETMBTOEL_kWh_ovrdflg
      link override Signal_Override/_ovrdval: Value=KOUTP_ETMBTOEL_kWh_ovrdval
  VDID_ETMBTOER_kWh_Inproc : FVT_lib/outp/OverrideAndLimit  SystemSampleTime=-1  VariantActivationTime=update diagram  Latency=0  AutoFrameSizeCalculation=off
      link override Signal_Limit/_maxval: Value=KOUTP_ETMBTOER_kWh_maxval
      link override Signal_Limit/_minval: Value=KOUTP_ETMBTOER_kWh_minval
      link override Signal_Override/_ovrdflg: Value=KOUTP_ETMBTOER_kWh_ovrdflg
      link override Signal_Override/_ovrdval: Value=KOUTP_ETMBTOER_kWh_ovrdval
  VDID_GECHGOVCACL_kWh_Inproc : FVT_lib/outp/OverrideAndLimit  SystemSampleTime=-1  VariantActivationTime=update diagram  Latency=0  AutoFrameSizeCalculation=off
      link override Signal_Limit/_maxval: Value=KOUTP_GECHGOVCACL_kWh_maxval
      link override Signal_Limit/_minval: Value=KOUTP_GECHGOVCACL_kWh_minval
      link override Signal_Override/_ovrdflg: Value=KOUTP_GECHGOVCACL_kWh_ovrdflg
      link override Signal_Override/_ovrdval: Value=KOUTP_GECHGOVCACL_kWh_ovrdval
  VDID_GECHGOVCACR_kWh_Inproc : FVT_lib/outp/OverrideAndLimit  SystemSampleTime=-1  VariantActivationTime=update diagram  Latency=0  AutoFrameSizeCalculation=off
      link override Signal_Limit/_maxval: Value=KOUTP_GECHGOVCACR_kWh_maxval
      link override Signal_Limit/_minval: Value=KOUTP_GECHGOVCACR_kWh_minval
      link override Signal_Override/_ovrdflg: Value=KOUTP_GECHGOVCACR_kWh_ovrdflg
      link override Signal_Override/_ovrdval: Value=KOUTP_GECHGOVCACR_kWh_ovrdval
  VDID_GECHGOVCDCL_kWh_Inproc : FVT_lib/outp/OverrideAndLimit  SystemSampleTime=-1  VariantActivationTime=update diagram  Latency=0  AutoFrameSizeCalculation=off
      link override Signal_Limit/_maxval: Value=KOUTP_GECHGOVCDCL_kWh_maxval
      link override Signal_Limit/_minval: Value=KOUTP_GECHGOVCDCL_kWh_minval
      link override Signal_Override/_ovrdflg: Value=KOUTP_GECHGOVCDCL_kWh_ovrdflg
      link override Signal_Override/_ovrdval: Value=KOUTP_GECHGOVCDCL_kWh_ovrdval
  VDID_GECHGOVCDCR_kWh_Inproc : FVT_lib/outp/OverrideAndLimit  SystemSampleTime=-1  VariantActivationTime=update diagram  Latency=0  AutoFrameSizeCalculation=off
      link override Signal_Limit/_maxval: Value=KOUTP_GECHGOVCDCR_kWh_maxval
      link override Signal_Limit/_minval: Value=KOUTP_GECHGOVCDCR_kWh_minval
      link override Signal_Override/_ovrdflg: Value=KOUTP_GECHGOVCDCR_kWh_ovrdflg
      link override Signal_Override/_ovrdval: Value=KOUTP_GECHGOVCDCR_kWh_ovrdval
  VDID_HEVBATT_V_Inproc : FVT_lib/outp/OverrideAndLimit  SystemSampleTime=-1  VariantActivationTime=update diagram  Latency=0  AutoFrameSizeCalculation=off
      link override Signal_Limit/_maxval: Value=KOUTP_HEVBATT_V_maxval
      link override Signal_Limit/_minval: Value=KOUTP_HEVBATT_V_minval
      link override Signal_Override/_ovrdflg: Value=KOUTP_HEVBATT_V_ovrdflg
      link override Signal_Override/_ovrdval: Value=KOUTP_HEVBATT_V_ovrdval
  VDID_HEVMODE_enum_Inproc : FVT_lib/outp/OverrideAndLimit  SystemSampleTime=-1  VariantActivationTime=update diagram  Latency=0  AutoFrameSizeCalculation=off
      link override Signal_Limit/_maxval: Value=KOUTP_HEVMODE_enum_maxval
      link override Signal_Limit/_minval: Value=KOUTP_HEVMODE_enum_minval
      link override Signal_Override/_ovrdflg: Value=KOUTP_HEVMODE_enum_ovrdflg
      link override Signal_Override/_ovrdval: Value=KOUTP_HEVMODE_enum_ovrdval
  VDID_HVBATT_A_Inproc : FVT_lib/outp/OverrideAndLimit  SystemSampleTime=-1  VariantActivationTime=update diagram  Latency=0  AutoFrameSizeCalculation=off
      link override Signal_Limit/_maxval: Value=KOUTP_HVBATT_A_maxval
      link override Signal_Limit/_minval: Value=KOUTP_HVBATT_A_minval
      link override Signal_Override/_ovrdflg: Value=KOUTP_HVBATT_A_ovrdflg
      link override Signal_Override/_ovrdval: Value=KOUTP_HVBATT_A_ovrdval
  VDID_HVBCellVoltMax_V_Inproc : FVT_lib/outp/OverrideAndLimit  SystemSampleTime=-1  VariantActivationTime=update diagram  Latency=0  AutoFrameSizeCalculation=off
      link override Signal_Limit/_maxval: Value=KOUTP_HVBCellVoltMax_V_maxval
      link override Signal_Limit/_minval: Value=KOUTP_HVBCellVoltMax_V_minval
      link override Signal_Override/_ovrdflg: Value=KOUTP_HVBCellVoltMax_V_ovrdflg
      link override Signal_Override/_ovrdval: Value=KOUTP_HVBCellVoltMax_V_ovrdval
  VDID_HVBCellVoltMin_V_Inproc : FVT_lib/outp/OverrideAndLimit  SystemSampleTime=-1  VariantActivationTime=update diagram  Latency=0  AutoFrameSizeCalculation=off
      link override Signal_Limit/_maxval: Value=KOUTP_HVBCellVoltMin_V_maxval
      link override Signal_Limit/_minval: Value=KOUTP_HVBCellVoltMin_V_minval
      link override Signal_Override/_ovrdflg: Value=KOUTP_HVBCellVoltMin_V_ovrdflg
      link override Signal_Override/_ovrdval: Value=KOUTP_HVBCellVoltMin_V_ovrdval
  VDID_HVBNAH_Ahr_Inproc : FVT_lib/outp/OverrideAndLimit  SystemSampleTime=-1  VariantActivationTime=update diagram  Latency=0  AutoFrameSizeCalculation=off
      link override Signal_Limit/_maxval: Value=KOUTP_HVBNAH_Ahr_maxval
      link override Signal_Limit/_minval: Value=KOUTP_HVBNAH_Ahr_minval
      link override Signal_Override/_ovrdflg: Value=KOUTP_HVBNAH_Ahr_ovrdflg
      link override Signal_Override/_ovrdval: Value=KOUTP_HVBNAH_Ahr_ovrdval
  VDID_HVBNE_kWh_Inproc : FVT_lib/outp/OverrideAndLimit  SystemSampleTime=-1  VariantActivationTime=update diagram  Latency=0  AutoFrameSizeCalculation=off
      link override Signal_Limit/_maxval: Value=KOUTP_HVBNE_kWh_maxval
      link override Signal_Limit/_minval: Value=KOUTP_HVBNE_kWh_minval
      link override Signal_Override/_ovrdflg: Value=KOUTP_HVBNE_kWh_ovrdflg
      link override Signal_Override/_ovrdval: Value=KOUTP_HVBNE_kWh_ovrdval
  VDID_HVBattCurr_Ahps_Inproc : FVT_lib/outp/OverrideAndLimit  SystemSampleTime=-1  VariantActivationTime=update diagram  Latency=0  AutoFrameSizeCalculation=off
      link override Signal_Limit/_maxval: Value=KOUTP_HVBattCurr_Ahps_maxval
      link override Signal_Limit/_minval: Value=KOUTP_HVBattCurr_Ahps_minval
      link override Signal_Override/_ovrdflg: Value=KOUTP_HVBattCurr_Ahps_ovrdflg
      link override Signal_Override/_ovrdval: Value=KOUTP_HVBattCurr_Ahps_ovrdval
  VDID_HVESSCHARGEACT_kW_Inproc : FVT_lib/outp/OverrideAndLimit  SystemSampleTime=-1  VariantActivationTime=update diagram  Latency=0  AutoFrameSizeCalculation=off
      link override Signal_Limit/_maxval: Value=KOUTP_HVESSCHARGEACT_kW_maxval
      link override Signal_Limit/_minval: Value=KOUTP_HVESSCHARGEACT_kW_minval
      link override Signal_Override/_ovrdflg: Value=KOUTP_HVESSCHARGEACT_kW_ovrdflg
      link override Signal_Override/_ovrdval: Value=KOUTP_HVESSCHARGEACT_kW_ovrdval
  VDID_HVESSCHARGELIM_kW_Inproc : FVT_lib/outp/OverrideAndLimit  SystemSampleTime=-1  VariantActivationTime=update diagram  Latency=0  AutoFrameSizeCalculation=off
      link override Signal_Limit/_maxval: Value=KOUTP_HVESSCHARGELIM_kW_maxval
      link override Signal_Limit/_minval: Value=KOUTP_HVESSCHARGELIM_kW_minval
      link override Signal_Override/_ovrdflg: Value=KOUTP_HVESSCHARGELIM_kW_ovrdflg
      link override Signal_Override/_ovrdval: Value=KOUTP_HVESSCHARGELIM_kW_ovrdval
  VDID_HVESSENER_Whps_Inproc : FVT_lib/outp/OverrideAndLimit  SystemSampleTime=-1  VariantActivationTime=update diagram  Latency=0  AutoFrameSizeCalculation=off
      link override Signal_Limit/_maxval: Value=KOUTP_HVESSENER_Whps_maxval
      link override Signal_Limit/_minval: Value=KOUTP_HVESSENER_Whps_minval
      link override Signal_Override/_ovrdflg: Value=KOUTP_HVESSENER_Whps_ovrdflg
      link override Signal_Override/_ovrdval: Value=KOUTP_HVESSENER_Whps_ovrdval
  VDID_IGNCNTR_cnt_Inproc : FVT_lib/outp/OverrideAndLimit  SystemSampleTime=-1  VariantActivationTime=update diagram  Latency=0  AutoFrameSizeCalculation=off
      link override Signal_Limit/_maxval: Value=KOUTP_IGNCNTR_cnt_maxval
      link override Signal_Limit/_minval: Value=KOUTP_IGNCNTR_cnt_minval
      link override Signal_Override/_ovrdflg: Value=KOUTP_IGNCNTR_cnt_ovrdflg
      link override Signal_Override/_ovrdval: Value=KOUTP_IGNCNTR_cnt_ovrdval
  VDID_IPSAL_sec_Inproc : FVT_lib/outp/OverrideAndLimit  SystemSampleTime=-1  VariantActivationTime=update diagram  Latency=0  AutoFrameSizeCalculation=off
      link override Signal_Limit/_maxval: Value=KOUTP_IPSAL_sec_maxval
      link override Signal_Limit/_minval: Value=KOUTP_IPSAL_sec_minval
      link override Signal_Override/_ovrdflg: Value=KOUTP_IPSAL_sec_ovrdflg
      link override Signal_Override/_ovrdval: Value=KOUTP_IPSAL_sec_ovrdval
  VDID_IPSAR_sec_Inproc : FVT_lib/outp/OverrideAndLimit  SystemSampleTime=-1  VariantActivationTime=update diagram  Latency=0  AutoFrameSizeCalculation=off
      link override Signal_Limit/_maxval: Value=KOUTP_IPSAR_sec_maxval
      link override Signal_Limit/_minval: Value=KOUTP_IPSAR_sec_minval
      link override Signal_Override/_ovrdflg: Value=KOUTP_IPSAR_sec_ovrdflg
      link override Signal_Override/_ovrdval: Value=KOUTP_IPSAR_sec_ovrdval
  VDID_MAXBATTEMPL_C_Inproc : FVT_lib/outp/OverrideAndLimit  SystemSampleTime=-1  VariantActivationTime=update diagram  Latency=0  AutoFrameSizeCalculation=off
      link override Signal_Limit/_maxval: Value=KOUTP_MAXBATTEMPL_C_maxval
      link override Signal_Limit/_minval: Value=KOUTP_MAXBATTEMPL_C_minval
      link override Signal_Override/_ovrdflg: Value=KOUTP_MAXBATTEMPL_C_ovrdflg
      link override Signal_Override/_ovrdval: Value=KOUTP_MAXBATTEMPL_C_ovrdval
  VDID_MILDIST_km_Inproc : FVT_lib/outp/OverrideAndLimit  SystemSampleTime=-1  VariantActivationTime=update diagram  Latency=0  AutoFrameSizeCalculation=off
      link override Signal_Limit/_maxval: Value=KOUTP_MILDIST_km_maxval
      link override Signal_Limit/_minval: Value=KOUTP_MILDIST_km_minval
      link override Signal_Override/_ovrdflg: Value=KOUTP_MILDIST_km_ovrdflg
      link override Signal_Override/_ovrdval: Value=KOUTP_MILDIST_km_ovrdval
  VDID_MILTIME_min_Inproc : FVT_lib/outp/OverrideAndLimit  SystemSampleTime=-1  VariantActivationTime=update diagram  Latency=0  AutoFrameSizeCalculation=off
      link override Signal_Limit/_maxval: Value=KOUTP_MILTIME_min_maxval
      link override Signal_Limit/_minval: Value=KOUTP_MILTIME_min_minval
      link override Signal_Override/_ovrdflg: Value=KOUTP_MILTIME_min_ovrdflg
      link override Signal_Override/_ovrdval: Value=KOUTP_MILTIME_min_ovrdval
  VDID_MINBATTEMPL_C_Inproc : FVT_lib/outp/OverrideAndLimit  SystemSampleTime=-1  VariantActivationTime=update diagram  Latency=0  AutoFrameSizeCalculation=off
      link override Signal_Limit/_maxval: Value=KOUTP_MINBATTEMPL_C_maxval
      link override Signal_Limit/_minval: Value=KOUTP_MINBATTEMPL_C_minval
      link override Signal_Override/_ovrdflg: Value=KOUTP_MINBATTEMPL_C_ovrdflg
      link override Signal_Override/_ovrdval: Value=KOUTP_MINBATTEMPL_C_ovrdval
  VDID_NUMPSATRIPSFLTMEMCLR_cnt_Inproc : FVT_lib/outp/OverrideAndLimit  SystemSampleTime=-1  VariantActivationTime=update diagram  Latency=0  AutoFrameSizeCalculation=off
      link override Signal_Limit/_maxval: Value=KOUTP_NUMPSATRIPSFLTMEMCLR_cnt_maxval
      link override Signal_Limit/_minval: Value=KOUTP_NUMPSATRIPSFLTMEMCLR_cnt_minval
      link override Signal_Override/_ovrdflg: Value=KOUTP_NUMPSATRIPSFLTMEMCLR_cnt_ovrdflg
      link override Signal_Override/_ovrdval: Value=KOUTP_NUMPSATRIPSFLTMEMCLR_cnt_ovrdval
  VDID_ODOMETER_km_Inproc : FVT_lib/outp/OverrideAndLimit  SystemSampleTime=-1  VariantActivationTime=update diagram  Latency=0  AutoFrameSizeCalculation=off
      link override Signal_Limit/_maxval: Value=KOUTP_ODOMETER_km_maxval
      link override Signal_Limit/_minval: Value=KOUTP_ODOMETER_km_minval
      link override Signal_Override/_ovrdflg: Value=KOUTP_ODOMETER_km_ovrdflg
      link override Signal_Override/_ovrdval: Value=KOUTP_ODOMETER_km_ovrdval
  VDID_OFFL_sec_Inproc : FVT_lib/outp/OverrideAndLimit  SystemSampleTime=-1  VariantActivationTime=update diagram  Latency=0  AutoFrameSizeCalculation=off
      link override Signal_Limit/_maxval: Value=KOUTP_OFFL_sec_maxval
      link override Signal_Limit/_minval: Value=KOUTP_OFFL_sec_minval
      link override Signal_Override/_ovrdflg: Value=KOUTP_OFFL_sec_ovrdflg
      link override Signal_Override/_ovrdval: Value=KOUTP_OFFL_sec_ovrdval
  VDID_OFFR_sec_Inproc : FVT_lib/outp/OverrideAndLimit  SystemSampleTime=-1  VariantActivationTime=update diagram  Latency=0  AutoFrameSizeCalculation=off
      link override Signal_Limit/_maxval: Value=KOUTP_OFFR_sec_maxval
      link override Signal_Limit/_minval: Value=KOUTP_OFFR_sec_minval
      link override Signal_Override/_ovrdflg: Value=KOUTP_OFFR_sec_ovrdflg
      link override Signal_Override/_ovrdval: Value=KOUTP_OFFR_sec_ovrdval
  VDID_OVCL_sec_Inproc : FVT_lib/outp/OverrideAndLimit  SystemSampleTime=-1  VariantActivationTime=update diagram  Latency=0  AutoFrameSizeCalculation=off
      link override Signal_Limit/_maxval: Value=KOUTP_OVCL_sec_maxval
      link override Signal_Limit/_minval: Value=KOUTP_OVCL_sec_minval
      link override Signal_Override/_ovrdflg: Value=KOUTP_OVCL_sec_ovrdflg
      link override Signal_Override/_ovrdval: Value=KOUTP_OVCL_sec_ovrdval
  VDID_OVCR_sec_Inproc : FVT_lib/outp/OverrideAndLimit  SystemSampleTime=-1  VariantActivationTime=update diagram  Latency=0  AutoFrameSizeCalculation=off
      link override Signal_Limit/_maxval: Value=KOUTP_OVCR_sec_maxval
      link override Signal_Limit/_minval: Value=KOUTP_OVCR_sec_minval
      link override Signal_Override/_ovrdflg: Value=KOUTP_OVCR_sec_ovrdflg
      link override Signal_Override/_ovrdval: Value=KOUTP_OVCR_sec_ovrdval
  VDID_PKELNumerator_kphsqr_Inproc : FVT_lib/outp/OverrideAndLimit  SystemSampleTime=-1  VariantActivationTime=update diagram  Latency=0  AutoFrameSizeCalculation=off
      link override Signal_Limit/_maxval: Value=KOUTP_PKELNumerator_kphsqr_maxval
      link override Signal_Limit/_minval: Value=KOUTP_PKELNumerator_kphsqr_minval
      link override Signal_Override/_ovrdflg: Value=KOUTP_PKELNumerator_kphsqr_ovrdflg
      link override Signal_Override/_ovrdval: Value=KOUTP_PKELNumerator_kphsqr_ovrdval
  VDID_PKEL_kphsqr_Inproc : FVT_lib/outp/OverrideAndLimit  SystemSampleTime=-1  VariantActivationTime=update diagram  Latency=0  AutoFrameSizeCalculation=off
      link override Signal_Limit/_maxval: Value=KOUTP_PKEL_kphsqr_maxval
      link override Signal_Limit/_minval: Value=KOUTP_PKEL_kphsqr_minval
      link override Signal_Override/_ovrdflg: Value=KOUTP_PKEL_kphsqr_ovrdflg
      link override Signal_Override/_ovrdval: Value=KOUTP_PKEL_kphsqr_ovrdval
  VDID_PKERNumerator_kphsqr_Inproc : FVT_lib/outp/OverrideAndLimit  SystemSampleTime=-1  VariantActivationTime=update diagram  Latency=0  AutoFrameSizeCalculation=off
      link override Signal_Limit/_maxval: Value=KOUTP_PKERNumerator_kphsqr_maxval
      link override Signal_Limit/_minval: Value=KOUTP_PKERNumerator_kphsqr_minval
      link override Signal_Override/_ovrdflg: Value=KOUTP_PKERNumerator_kphsqr_ovrdflg
      link override Signal_Override/_ovrdval: Value=KOUTP_PKERNumerator_kphsqr_ovrdval
  VDID_PKER_kphsqr_Inproc : FVT_lib/outp/OverrideAndLimit  SystemSampleTime=-1  VariantActivationTime=update diagram  Latency=0  AutoFrameSizeCalculation=off
      link override Signal_Limit/_maxval: Value=KOUTP_PKER_kphsqr_maxval
      link override Signal_Limit/_minval: Value=KOUTP_PKER_kphsqr_minval
      link override Signal_Override/_ovrdflg: Value=KOUTP_PKER_kphsqr_ovrdflg
      link override Signal_Override/_ovrdval: Value=KOUTP_PKER_kphsqr_ovrdval
  VDID_PROTOCOLID_enum_Inproc : FVT_lib/outp/OverrideAndLimit  SystemSampleTime=-1  VariantActivationTime=update diagram  Latency=0  AutoFrameSizeCalculation=off
      link override Signal_Limit/_maxval: Value=KOUTP_PROTOCOLID_enum_maxval
      link override Signal_Limit/_minval: Value=KOUTP_PROTOCOLID_enum_minval
      link override Signal_Override/_ovrdflg: Value=KOUTP_PROTOCOLID_enum_ovrdflg
      link override Signal_Override/_ovrdval: Value=KOUTP_PROTOCOLID_enum_ovrdval
  VDID_PSAL_sec_Inproc : FVT_lib/outp/OverrideAndLimit  SystemSampleTime=-1  VariantActivationTime=update diagram  Latency=0  AutoFrameSizeCalculation=off
      link override Signal_Limit/_maxval: Value=KOUTP_PSAL_sec_maxval
      link override Signal_Limit/_minval: Value=KOUTP_PSAL_sec_minval
      link override Signal_Override/_ovrdflg: Value=KOUTP_PSAL_sec_ovrdflg
      link override Signal_Override/_ovrdval: Value=KOUTP_PSAL_sec_ovrdval
  VDID_PSAR_sec_Inproc : FVT_lib/outp/OverrideAndLimit  SystemSampleTime=-1  VariantActivationTime=update diagram  Latency=0  AutoFrameSizeCalculation=off
      link override Signal_Limit/_maxval: Value=KOUTP_PSAR_sec_maxval
      link override Signal_Limit/_minval: Value=KOUTP_PSAR_sec_minval
      link override Signal_Override/_ovrdflg: Value=KOUTP_PSAR_sec_ovrdflg
      link override Signal_Override/_ovrdval: Value=KOUTP_PSAR_sec_ovrdval
  VDID_QTYPSATRIPSL_cnt_Inproc : FVT_lib/outp/OverrideAndLimit  SystemSampleTime=-1  VariantActivationTime=update diagram  Latency=0  AutoFrameSizeCalculation=off
      link override Signal_Limit/_maxval: Value=KOUTP_QTYPSATRIPSL_cnt_maxval
      link override Signal_Limit/_minval: Value=KOUTP_QTYPSATRIPSL_cnt_minval
      link override Signal_Override/_ovrdflg: Value=KOUTP_QTYPSATRIPSL_cnt_ovrdflg
      link override Signal_Override/_ovrdval: Value=KOUTP_QTYPSATRIPSL_cnt_ovrdval
  VDID_QTYPSATRIPSR_cnt_Inproc : FVT_lib/outp/OverrideAndLimit  SystemSampleTime=-1  VariantActivationTime=update diagram  Latency=0  AutoFrameSizeCalculation=off
      link override Signal_Limit/_maxval: Value=KOUTP_QTYPSATRIPSR_cnt_maxval
      link override Signal_Limit/_minval: Value=KOUTP_QTYPSATRIPSR_cnt_minval
      link override Signal_Override/_ovrdflg: Value=KOUTP_QTYPSATRIPSR_cnt_ovrdflg
      link override Signal_Override/_ovrdval: Value=KOUTP_QTYPSATRIPSR_cnt_ovrdval
  VDID_RESSCNTDODRNGL_cnt_Inproc : FVT_lib/outp/OverrideAndLimit  SystemSampleTime=-1  VariantActivationTime=update diagram  Latency=0  AutoFrameSizeCalculation=off
      link override Signal_Limit/_maxval: Value=KOUTP_RESSCNTDODRNGL_cnt_maxval
      link override Signal_Limit/_minval: Value=KOUTP_RESSCNTDODRNGL_cnt_minval
      link override Signal_Override/_ovrdflg: Value=KOUTP_RESSCNTDODRNGL_cnt_ovrdflg
      link override Signal_Override/_ovrdval: Value=KOUTP_RESSCNTDODRNGL_cnt_ovrdval
  VDID_RESSCNTDODRNGR_cnt_Inproc : FVT_lib/outp/OverrideAndLimit  SystemSampleTime=-1  VariantActivationTime=update diagram  Latency=0  AutoFrameSizeCalculation=off
      link override Signal_Limit/_maxval: Value=KOUTP_RESSCNTDODRNGR_cnt_maxval
      link override Signal_Limit/_minval: Value=KOUTP_RESSCNTDODRNGR_cnt_minval
      link override Signal_Override/_ovrdflg: Value=KOUTP_RESSCNTDODRNGR_cnt_ovrdflg
      link override Signal_Override/_ovrdval: Value=KOUTP_RESSCNTDODRNGR_cnt_ovrdval
  VDID_RESSCNTSDODRNGAXIS_enum_Inproc : FVT_lib/outp/OverrideAndLimit  SystemSampleTime=-1  VariantActivationTime=update diagram  Latency=0  AutoFrameSizeCalculation=off
      link override Signal_Limit/_maxval: Value=KOUTP_RESSCNTSDODRNGAXIS_enum_maxval
      link override Signal_Limit/_minval: Value=KOUTP_RESSCNTSDODRNGAXIS_enum_minval
      link override Signal_Override/_ovrdflg: Value=KOUTP_RESSCNTSDODRNGAXIS_enum_ovrdflg
      link override Signal_Override/_ovrdval: Value=KOUTP_RESSCNTSDODRNGAXIS_enum_ovrdval
  VDID_RESSTIMESOCCHGRNGL_s_Inproc : FVT_lib/outp/OverrideAndLimit  SystemSampleTime=-1  VariantActivationTime=update diagram  Latency=0  AutoFrameSizeCalculation=off
      link override Signal_Limit/_maxval: Value=KOUTP_RESSTIMESOCCHGRNGL_s_maxval
      link override Signal_Limit/_minval: Value=KOUTP_RESSTIMESOCCHGRNGL_s_minval
      link override Signal_Override/_ovrdflg: Value=KOUTP_RESSTIMESOCCHGRNGL_s_ovrdflg
      link override Signal_Override/_ovrdval: Value=KOUTP_RESSTIMESOCCHGRNGL_s_ovrdval
  VDID_RESSTIMESOCCHGRNGR_s_Inproc : FVT_lib/outp/OverrideAndLimit  SystemSampleTime=-1  VariantActivationTime=update diagram  Latency=0  AutoFrameSizeCalculation=off
      link override Signal_Limit/_maxval: Value=KOUTP_RESSTIMESOCCHGRNGR_s_maxval
      link override Signal_Limit/_minval: Value=KOUTP_RESSTIMESOCCHGRNGR_s_minval
      link override Signal_Override/_ovrdflg: Value=KOUTP_RESSTIMESOCCHGRNGR_s_ovrdflg
      link override Signal_Override/_ovrdval: Value=KOUTP_RESSTIMESOCCHGRNGR_s_ovrdval
  VDID_RESSTIMESOCOFFRNGL_s_Inproc : FVT_lib/outp/OverrideAndLimit  SystemSampleTime=-1  VariantActivationTime=update diagram  Latency=0  AutoFrameSizeCalculation=off
      link override Signal_Limit/_maxval: Value=KOUTP_RESSTIMESOCOFFRNGL_s_maxval
      link override Signal_Limit/_minval: Value=KOUTP_RESSTIMESOCOFFRNGL_s_minval
      link override Signal_Override/_ovrdflg: Value=KOUTP_RESSTIMESOCOFFRNGL_s_ovrdflg
      link override Signal_Override/_ovrdval: Value=KOUTP_RESSTIMESOCOFFRNGL_s_ovrdval
  VDID_RESSTIMESOCOFFRNGR_s_Inproc : FVT_lib/outp/OverrideAndLimit  SystemSampleTime=-1  VariantActivationTime=update diagram  Latency=0  AutoFrameSizeCalculation=off
      link override Signal_Limit/_maxval: Value=KOUTP_RESSTIMESOCOFFRNGR_s_maxval
      link override Signal_Limit/_minval: Value=KOUTP_RESSTIMESOCOFFRNGR_s_minval
      link override Signal_Override/_ovrdflg: Value=KOUTP_RESSTIMESOCOFFRNGR_s_ovrdflg
      link override Signal_Override/_ovrdval: Value=KOUTP_RESSTIMESOCOFFRNGR_s_ovrdval
  VDID_RESSTIMESOCPSARNGL_s_Inproc : FVT_lib/outp/OverrideAndLimit  SystemSampleTime=-1  VariantActivationTime=update diagram  Latency=0  AutoFrameSizeCalculation=off
      link override Signal_Limit/_maxval: Value=KOUTP_RESSTIMESOCPSARNGL_s_maxval
      link override Signal_Limit/_minval: Value=KOUTP_RESSTIMESOCPSARNGL_s_minval
      link override Signal_Override/_ovrdflg: Value=KOUTP_RESSTIMESOCPSARNGL_s_ovrdflg
      link override Signal_Override/_ovrdval: Value=KOUTP_RESSTIMESOCPSARNGL_s_ovrdval
  VDID_RESSTIMESOCPSARNGR_s_Inproc : FVT_lib/outp/OverrideAndLimit  SystemSampleTime=-1  VariantActivationTime=update diagram  Latency=0  AutoFrameSizeCalculation=off
      link override Signal_Limit/_maxval: Value=KOUTP_RESSTIMESOCPSARNGR_s_maxval
      link override Signal_Limit/_minval: Value=KOUTP_RESSTIMESOCPSARNGR_s_minval
      link override Signal_Override/_ovrdflg: Value=KOUTP_RESSTIMESOCPSARNGR_s_ovrdflg
      link override Signal_Override/_ovrdval: Value=KOUTP_RESSTIMESOCPSARNGR_s_ovrdval
  VDID_RESSTIMESOCRNGAXIS_enum_Inproc : FVT_lib/outp/OverrideAndLimit  SystemSampleTime=-1  VariantActivationTime=update diagram  Latency=0  AutoFrameSizeCalculation=off
      link override Signal_Limit/_maxval: Value=KOUTP_RESSTIMESOCRNGAXIS_enum_maxval
      link override Signal_Limit/_minval: Value=KOUTP_RESSTIMESOCRNGAXIS_enum_minval
      link override Signal_Override/_ovrdflg: Value=KOUTP_RESSTIMESOCRNGAXIS_enum_ovrdflg
      link override Signal_Override/_ovrdval: Value=KOUTP_RESSTIMESOCRNGAXIS_enum_ovrdval
  VDID_RESSTTEMPRNGAXIS_enum_Inproc : FVT_lib/outp/OverrideAndLimit  SystemSampleTime=-1  VariantActivationTime=update diagram  Latency=0  AutoFrameSizeCalculation=off
      link override Signal_Limit/_maxval: Value=KOUTP_RESSTTEMPRNGAXIS_enum_maxval
      link override Signal_Limit/_minval: Value=KOUTP_RESSTTEMPRNGAXIS_enum_minval
      link override Signal_Override/_ovrdflg: Value=KOUTP_RESSTTEMPRNGAXIS_enum_ovrdflg
      link override Signal_Override/_ovrdval: Value=KOUTP_RESSTTEMPRNGAXIS_enum_ovrdval
  VDID_RESSV2XENNONPSAL_kWh_Inproc : FVT_lib/outp/OverrideAndLimit  SystemSampleTime=-1  VariantActivationTime=update diagram  Latency=0  AutoFrameSizeCalculation=off
      link override Signal_Limit/_maxval: Value=KOUTP_RESSV2XENNONPSAL_kWh_maxval
      link override Signal_Limit/_minval: Value=KOUTP_RESSV2XENNONPSAL_kWh_minval
      link override Signal_Override/_ovrdflg: Value=KOUTP_RESSV2XENNONPSAL_kWh_ovrdflg
      link override Signal_Override/_ovrdval: Value=KOUTP_RESSV2XENNONPSAL_kWh_ovrdval
  VDID_RESSV2XENNONPSAR_kWh_Inproc : FVT_lib/outp/OverrideAndLimit  SystemSampleTime=-1  VariantActivationTime=update diagram  Latency=0  AutoFrameSizeCalculation=off
      link override Signal_Limit/_maxval: Value=KOUTP_RESSV2XENNONPSAR_kWh_maxval
      link override Signal_Limit/_minval: Value=KOUTP_RESSV2XENNONPSAR_kWh_minval
      link override Signal_Override/_ovrdflg: Value=KOUTP_RESSV2XENNONPSAR_kWh_ovrdflg
      link override Signal_Override/_ovrdval: Value=KOUTP_RESSV2XENNONPSAR_kWh_ovrdval
  VDID_RUNTM_s_Inproc : FVT_lib/outp/OverrideAndLimit  SystemSampleTime=-1  VariantActivationTime=update diagram  Latency=0  AutoFrameSizeCalculation=off
      link override Signal_Limit/_maxval: Value=KOUTP_RUNTM_s_maxval
      link override Signal_Limit/_minval: Value=KOUTP_RUNTM_s_minval
